simulink model "TrackingAdaptiveTaskSpace"  (R2019a)
settings: Solver=ode23  StartTime=0.0  StopTime=10  FixedStep=0.01  RelTol=1e-4
libraries: dspmtrx3 x3, dspinverses x1
(part 2 of 2)

== matlab function TrackingAdaptiveTaskSpace/MATLAB Function1 ==
  data: q1 input; aux output; q2 input; q3 input; q4 input; L1 input; L2 input; L3 input; L4 input
function aux = fcn(q1,q2,q3,q4,L1,L2,L3,L4)
%%%
aux11 = 0;
aux21 = (0.5000*(L2*L4*cos(conj(q1))*cos(conj(q1) + conj(q2) + conj(q3))*cos(q1 + q2 + q3 + q4)*conj(L1)*conj(L3)*sin(q1 + q2) - L2*L4*cos(conj(q1))*cos(conj(q1) + conj(q2) + conj(q3))*sin(q1 + q2 + q3 + q4)*cos(q1 + q2)*conj(L1)*conj(L3) + 3*L1*L4*cos(conj(q1) + conj(q2) + conj(q3) + conj(q4))*cos(conj(q1))*cos(q1 + q2 + q3 + q4)*conj(L1)*conj(L4)*sin(q1) - 3*L1*L4*cos(conj(q1) + conj(q2) + conj(q3) + conj(q4))*cos(conj(q1))*sin(q1 + q2 + q3 + q4)*conj(L1)*conj(L4)*cos(q1) + 3*L1*L4*cos(conj(q1) + conj(q2) + conj(q3) + conj(q4))*sin(conj(q1))*cos(q1 + q2 + q3 + q4)*conj(L1)*conj(L4)*cos(q1) - 3*L1*L4*sin(conj(q1) + conj(q2) + conj(q3) + conj(q4))*cos(conj(q1))*cos(q1 + q2 + q3 + q4)*conj(L1)*conj(L4)*cos(q1) + L1*L3*cos(q1 + q2 + q3)*sin(conj(q1))*sin(conj(q1) + conj(q2))*conj(L1)*conj(L2)*sin(q1) - L1*L3*sin(q1 + q2 + q3)*cos(conj(q1))*sin(conj(q1) + conj(q2))*conj(L1)*conj(L2)*sin(q1) + L1*L3*sin(q1 + q2 + q3)*sin(conj(q1))*cos(conj(q1) + conj(q2))*conj(L1)*conj(L2)*sin(q1) - L1*L3*sin(q1 + q2 + q3)*sin(conj(q1))*sin(conj(q1) + conj(q2))*conj(L1)*conj(L2)*cos(q1) + L1*L4*cos(conj(q1) + conj(q2) + conj(q3) + conj(q4))*sin(conj(q1) + conj(q2) + conj(q3))*cos(q1 + q2 + q3 + q4)*conj(L3)*conj(L4)*cos(q1) - L1*L4*sin(conj(q1) + conj(q2) + conj(q3) + conj(q4))*cos(conj(q1) + conj(q2) + conj(q3))*cos(q1 + q2 + q3 + q4)*conj(L3)*conj(L4)*cos(q1) + L1*L3*sin(q1 + q2 + q3)*cos(conj(q1) + conj(q2) + conj(q3))*sin(conj(q1) + conj(q2))*conj(L2)*conj(L3)*sin(q1) - L1*L3*sin(q1 + q2 + q3)*sin(conj(q1) + conj(q2) + conj(q3))*cos(conj(q1) + conj(q2))*conj(L2)*conj(L3)*sin(q1) + L2*L4*sin(conj(q1))*sin(conj(q1) + conj(q2) + conj(q3))*cos(q1 + q2 + q3 + q4)*conj(L1)*conj(L3)*sin(q1 + q2) - L2*L4*sin(conj(q1))*sin(conj(q1) + conj(q2) + conj(q3))*sin(q1 + q2 + q3 + q4)*cos(q1 + q2)*conj(L1)*conj(L3) + L1*L2*cos(conj(q1) + conj(q2) + conj(q3) + conj(q4))*cos(conj(q1))*cos(q1 + q2)*conj(L1)*conj(L4)*sin(q1) - L1*L2*cos(conj(q1) + conj(q2) + conj(q3) + conj(q4))*cos(conj(q1))*conj(L1)*conj(L4)*sin(q1 + q2)*cos(q1) + L1*L2*cos(conj(q1) + conj(q2) + conj(q3) + conj(q4))*sin(conj(q1))*cos(q1 + q2)*conj(L1)*conj(L4)*cos(q1) - L1*L2*sin(conj(q1) + conj(q2) + conj(q3) + conj(q4))*cos(conj(q1))*cos(q1 + q2)*conj(L1)*conj(L4)*cos(q1) + 3*L1*L4*cos(conj(q1) + conj(q2) + conj(q3) + conj(q4))*sin(conj(q1))*sin(q1 + q2 + q3 + q4)*conj(L1)*conj(L4)*sin(q1) - 3*L1*L4*sin(conj(q1) + conj(q2) + conj(q3) + conj(q4))*cos(conj(q1))*sin(q1 + q2 + q3 + q4)*conj(L1)*conj(L4)*sin(q1) + 3*L1*L4*sin(conj(q1) + conj(q2) + conj(q3) + conj(q4))*sin(conj(q1))*cos(q1 + q2 + q3 + q4)*conj(L1)*conj(L4)*sin(q1) - 3*L1*L4*sin(conj(q1) + conj(q2) + conj(q3) + conj(q4))*sin(conj(q1))*sin(q1 + q2 + q3 + q4)*conj(L1)*conj(L4)*cos(q1) + L1*L4*cos(conj(q1) + conj(q2) + conj(q3) + conj(q4))*sin(conj(q1) + conj(q2) + conj(q3))*sin(q1 + q2 + q3 + q4)*conj(L3)*conj(L4)*sin(q1) - L1*L4*sin(conj(q1) + conj(q2) + conj(q3) + conj(q4))*cos(conj(q1) + conj(q2) + conj(q3))*sin(q1 + q2 + q3 + q4)*conj(L3)*conj(L4)*sin(q1) + 2*L1*L4*cos(conj(q1))*cos(conj(q1) + conj(q2) + conj(q3))*cos(q1 + q2 + q3 + q4)*conj(L1)*conj(L3)*sin(q1) - 2*L1*L4*cos(conj(q1))*cos(conj(q1) + conj(q2) + conj(q3))*sin(q1 + q2 + q3 + q4)*conj(L1)*conj(L3)*cos(q1) - 2*L1*L4*cos(conj(q1))*sin(conj(q1) + conj(q2) + conj(q3))*cos(q1 + q2 + q3 + q4)*conj(L1)*conj(L3)*cos(q1) + 2*L1*L4*cos(conj(q1) + conj(q2) + conj(q3))*sin(conj(q1))*cos(q1 + q2 + q3 + q4)*conj(L1)*conj(L3)*cos(q1) + 2*L1*L4*cos(conj(q1) + conj(q2) + conj(q3) + conj(q4))*sin(conj(q1) + conj(q2))*cos(q1 + q2 + q3 + q4)*conj(L2)*conj(L4)*cos(q1) - 2*L1*L4*sin(conj(q1) + conj(q2) + conj(q3) + conj(q4))*cos(conj(q1) + conj(q2))*cos(q1 + q2 + q3 + q4)*conj(L2)*conj(L4)*cos(q1) + L1*L2*cos(conj(q1) + conj(q2) + conj(q3) + conj(q4))*sin(conj(q1))*conj(L1)*conj(L4)*sin(q1 + q2)*sin(q1) - L1*L2*sin(conj(q1) + conj(q2) + conj(q3) + conj(q4))*cos(conj(q1))*conj(L1)*conj(L4)*sin(q1 + q2)*sin(q1) + L1*L2*sin(conj(q1) + conj(q2) + conj(q3) + conj(q4))*sin(conj(q1))*cos(q1 + q2)*conj(L1)*conj(L4)*sin(q1) - L1*L2*sin(conj(q1) + conj(q2) + conj(q3) + conj(q4))*sin(conj(q1))*conj(L1)*conj(L4)*sin(q1 + q2)*cos(q1) - L3*L4*cos(conj(q1) + conj(q2) + conj(q3) + conj(q4))*cos(q1 + q2 + q3)*cos(conj(q1))*sin(q1 + q2 + q3 + q4)*conj(L1)*conj(L4) + L3*L4*cos(conj(q1) + conj(q2) + conj(q3) + conj(q4))*sin(q1 + q2 + q3)*cos(conj(q1))*cos(q1 + q2 + q3 + q4)*conj(L1)*conj(L4) + L1*L2*cos(conj(q1))*cos(conj(q1) + conj(q2) + conj(q3))*cos(q1 + q2)*conj(L1)*conj(L3)*sin(q1) - L1*L2*cos(conj(q1))*cos(conj(q1) + conj(q2) + conj(q3))*conj(L1)*conj(L3)*sin(q1 + q2)*cos(q1) - L1*L2*cos(conj(q1))*sin(conj(q1) + conj(q2) + conj(q3))*cos(q1 + q2)*conj(L1)*conj(L3)*cos(q1) + L1*L2*cos(conj(q1) + conj(q2) + conj(q3))*sin(conj(q1))*cos(q1 + q2)*conj(L1)*conj(L3)*cos(q1) - 2*L1*L4*cos(conj(q1))*sin(conj(q1) + conj(q2) + conj(q3))*sin(q1 + q2 + q3 + q4)*conj(L1)*conj(L3)*sin(q1) + 2*L1*L4*cos(conj(q1) + conj(q2) + conj(q3))*sin(conj(q1))*sin(q1 + q2 + q3 + q4)*conj(L1)*conj(L3)*sin(q1) + 2*L1*L4*sin(conj(q1))*sin(conj(q1) + conj(q2) + conj(q3))*cos(q1 + q2 + q3 + q4)*conj(L1)*conj(L3)*sin(q1) - 2*L1*L4*sin(conj(q1))*sin(conj(q1) + conj(q2) + conj(q3))*sin(q1 + q2 + q3 + q4)*conj(L1)*conj(L3)*cos(q1) + 2*L1*L4*cos(conj(q1) + conj(q2) + conj(q3) + conj(q4))*sin(conj(q1) + conj(q2))*sin(q1 + q2 + q3 + q4)*conj(L2)*conj(L4)*sin(q1) - 2*L1*L4*sin(conj(q1) + conj(q2) + conj(q3) + conj(q4))*cos(conj(q1) + conj(q2))*sin(q1 + q2 + q3 + q4)*conj(L2)*conj(L4)*sin(q1) + L1*L4*cos(conj(q1))*cos(conj(q1) + conj(q2))*cos(q1 + q2 + q3 + q4)*conj(L1)*conj(L2)*sin(q1) - L1*L4*cos(conj(q1))*cos(conj(q1) + conj(q2))*sin(q1 + q2 + q3 + q4)*conj(L1)*conj(L2)*cos(q1) - L1*L4*cos(conj(q1))*sin(conj(q1) + conj(q2))*cos(q1 + q2 + q3 + q4)*conj(L1)*conj(L2)*cos(q1) + L1*L4*sin(conj(q1))*cos(conj(q1) + conj(q2))*cos(q1 + q2 + q3 + q4)*conj(L1)*conj(L2)*cos(q1) + L1*L4*cos(conj(q1) + conj(q2) + conj(q3))*sin(conj(q1) + conj(q2))*cos(q1 + q2 + q3 + q4)*conj(L2)*conj(L3)*cos(q1) - L1*L4*sin(conj(q1) + conj(q2) + conj(q3))*cos(conj(q1) + conj(q2))*cos(q1 + q2 + q3 + q4)*conj(L2)*conj(L3)*cos(q1) + L2*L3*cos(conj(q1) + conj(q2) + conj(q3) + conj(q4))*cos(q1 + q2 + q3)*cos(conj(q1))*conj(L1)*conj(L4)*sin(q1 + q2) - L2*L3*cos(conj(q1) + conj(q2) + conj(q3) + conj(q4))*sin(q1 + q2 + q3)*cos(conj(q1))*cos(q1 + q2)*conj(L1)*conj(L4) - L3*L4*cos(q1 + q2 + q3)*sin(conj(q1) + conj(q2) + conj(q3) + conj(q4))*sin(conj(q1))*sin(q1 + q2 + q3 + q4)*conj(L1)*conj(L4) + L3*L4*sin(conj(q1) + conj(q2) + conj(q3) + conj(q4))*sin(q1 + q2 + q3)*sin(conj(q1))*cos(q1 + q2 + q3 + q4)*conj(L1)*conj(L4) - L1*L2*cos(conj(q1))*sin(conj(q1) + conj(q2) + conj(q3))*conj(L1)*conj(L3)*sin(q1 + q2)*sin(q1) + L1*L2*cos(conj(q1) + conj(q2) + conj(q3))*sin(conj(q1))*conj(L1)*conj(L3)*sin(q1 + q2)*sin(q1) + L1*L2*sin(conj(q1))*sin(conj(q1) + conj(q2) + conj(q3))*cos(q1 + q2)*conj(L1)*conj(L3)*sin(q1) - L1*L2*sin(conj(q1))*sin(conj(q1) + conj(q2) + conj(q3))*conj(L1)*conj(L3)*sin(q1 + q2)*cos(q1) + L1*L2*cos(conj(q1))*cos(conj(q1) + conj(q2))*cos(q1 + q2)*conj(L1)*conj(L2)*sin(q1) - L1*L2*cos(conj(q1))*cos(conj(q1) + conj(q2))*conj(L1)*conj(L2)*sin(q1 + q2)*cos(q1) - L1*L2*cos(conj(q1))*sin(conj(q1) + conj(q2))*cos(q1 + q2)*conj(L1)*conj(L2)*cos(q1) + L1*L2*sin(conj(q1))*cos(conj(q1) + conj(q2))*cos(q1 + q2)*conj(L1)*conj(L2)*cos(q1) - L1*L4*cos(conj(q1))*sin(conj(q1) + conj(q2))*sin(q1 + q2 + q3 + q4)*conj(L1)*conj(L2)*sin(q1) + L1*L4*sin(conj(q1))*cos(conj(q1) + conj(q2))*sin(q1 + q2 + q3 + q4)*conj(L1)*conj(L2)*sin(q1) + L1*L4*sin(conj(q1))*sin(conj(q1) + conj(q2))*cos(q1 + q2 + q3 + q4)*conj(L1)*conj(L2)*sin(q1) - L1*L4*sin(conj(q1))*sin(conj(q1) + conj(q2))*sin(q1 + q2 + q3 + q4)*conj(L1)*conj(L2)*cos(q1) + L1*L4*cos(conj(q1) + conj(q2) + conj(q3))*sin(conj(q1) + conj(q2))*sin(q1 + q2 + q3 + q4)*conj(L2)*conj(L3)*sin(q1) - L1*L4*sin(conj(q1) + conj(q2) + conj(q3))*cos(conj(q1) + conj(q2))*sin(q1 + q2 + q3 + q4)*conj(L2)*conj(L3)*sin(q1) + L2*L3*cos(q1 + q2 + q3)*sin(conj(q1) + conj(q2) + conj(q3) + conj(q4))*sin(conj(q1))*conj(L1)*conj(L4)*sin(q1 + q2) - L2*L3*sin(conj(q1) + conj(q2) + conj(q3) + conj(q4))*sin(q1 + q2 + q3)*sin(conj(q1))*cos(q1 + q2)*conj(L1)*conj(L4) + L2*L3*cos(q1 + q2 + q3)*cos(conj(q1))*cos(conj(q1) + conj(q2) + conj(q3))*conj(L1)*conj(L3)*sin(q1 + q2) - L2*L3*sin(q1 + q2 + q3)*cos(conj(q1))*cos(conj(q1) + conj(q2) + conj(q3))*cos(q1 + q2)*conj(L1)*conj(L3) + 2*L1*L3*cos(conj(q1) + conj(q2) + conj(q3) + conj(q4))*cos(q1 + q2 + q3)*cos(conj(q1))*conj(L1)*conj(L4)*sin(q1) + 2*L1*L3*cos(conj(q1) + conj(q2) + conj(q3) + conj(q4))*cos(q1 + q2 + q3)*sin(conj(q1))*conj(L1)*conj(L4)*cos(q1) - 2*L1*L3*cos(conj(q1) + conj(q2) + conj(q3) + conj(q4))*sin(q1 + q2 + q3)*cos(conj(q1))*conj(L1)*conj(L4)*cos(q1) - 2*L1*L3*cos(q1 + q2 + q3)*sin(conj(q1) + conj(q2) + conj(q3) + conj(q4))*cos(conj(q1))*conj(L1)*conj(L4)*cos(q1) - L1*L2*cos(conj(q1))*sin(conj(q1) + conj(q2))*conj(L1)*conj(L2)*sin(q1 + q2)*sin(q1) + L1*L2*sin(conj(q1))*cos(conj(q1) + conj(q2))*conj(L1)*conj(L2)*sin(q1 + q2)*sin(q1) + L1*L2*sin(conj(q1))*sin(conj(q1) + conj(q2))*cos(q1 + q2)*conj(L1)*conj(L2)*sin(q1) - L1*L2*sin(conj(q1))*sin(conj(q1) + conj(q2))*conj(L1)*conj(L2)*sin(q1 + q2)*cos(q1) + L2*L3*cos(q1 + q2 + q3)*sin(conj(q1))*sin(conj(q1) + conj(q2) + conj(q3))*conj(L1)*conj(L3)*sin(q1 + q2) - L2*L3*sin(q1 + q2 + q3)*sin(conj(q1))*sin(conj(q1) + conj(q2) + conj(q3))*cos(q1 + q2)*conj(L1)*conj(L3) + 2*L1*L3*cos(conj(q1) + conj(q2) + conj(q3) + conj(q4))*sin(q1 + q2 + q3)*sin(conj(q1))*conj(L1)*conj(L4)*sin(q1) + 2*L1*L3*cos(q1 + q2 + q3)*sin(conj(q1) + conj(q2) + conj(q3) + conj(q4))*sin(conj(q1))*conj(L1)*conj(L4)*sin(q1) - 2*L1*L3*sin(conj(q1) + conj(q2) + conj(q3) + conj(q4))*sin(q1 + q2 + q3)*cos(conj(q1))*conj(L1)*conj(L4)*sin(q1) - 2*L1*L3*sin(conj(q1) + conj(q2) + conj(q3) + conj(q4))*sin(q1 + q2 + q3)*sin(conj(q1))*conj(L1)*conj(L4)*cos(q1) + 2*L1*L3*cos(q1 + q2 + q3)*cos(conj(q1))*cos(conj(q1) + conj(q2) + conj(q3))*conj(L1)*conj(L3)*sin(q1) - 2*L1*L3*cos(q1 + q2 + q3)*cos(conj(q1))*sin(conj(q1) + conj(q2) + conj(q3))*conj(L1)*conj(L3)*cos(q1) + 2*L1*L3*cos(q1 + q2 + q3)*cos(conj(q1) + conj(q2) + conj(q3))*sin(conj(q1))*conj(L1)*conj(L3)*cos(q1) - 2*L1*L3*sin(q1 + q2 + q3)*cos(conj(q1))*cos(conj(q1) + conj(q2) + conj(q3))*conj(L1)*conj(L3)*cos(q1) + L1*L3*cos(conj(q1) + conj(q2) + conj(q3) + conj(q4))*cos(q1 + q2 + q3)*sin(conj(q1) + conj(q2))*conj(L2)*conj(L4)*cos(q1) - L1*L3*cos(q1 + q2 + q3)*sin(conj(q1) + conj(q2) + conj(q3) + conj(q4))*cos(conj(q1) + conj(q2))*conj(L2)*conj(L4)*cos(q1) + 2*L2*L4*cos(conj(q1) + conj(q2) + conj(q3) + conj(q4))*cos(conj(q1))*cos(q1 + q2 + q3 + q4)*conj(L1)*conj(L4)*sin(q1 + q2) - 2*L2*L4*cos(conj(q1) + conj(q2) + conj(q3) + conj(q4))*cos(conj(q1))*sin(q1 + q2 + q3 + q4)*cos(q1 + q2)*conj(L1)*conj(L4) + 2*L1*L3*cos(q1 + q2 + q3)*sin(conj(q1))*sin(conj(q1) + conj(q2) + conj(q3))*conj(L1)*conj(L3)*sin(q1) - 2*L1*L3*sin(q1 + q2 + q3)*cos(conj(q1))*sin(conj(q1) + conj(q2) + conj(q3))*conj(L1)*conj(L3)*sin(q1) + 2*L1*L3*sin(q1 + q2 + q3)*cos(conj(q1) + conj(q2) + conj(q3))*sin(conj(q1))*conj(L1)*conj(L3)*sin(q1) - 2*L1*L3*sin(q1 + q2 + q3)*sin(conj(q1))*sin(conj(q1) + conj(q2) + conj(q3))*conj(L1)*conj(L3)*cos(q1) + L1*L3*cos(conj(q1) + conj(q2) + conj(q3) + conj(q4))*sin(q1 + q2 + q3)*sin(conj(q1) + conj(q2))*conj(L2)*conj(L4)*sin(q1) - L1*L3*sin(conj(q1) + conj(q2) + conj(q3) + conj(q4))*sin(q1 + q2 + q3)*cos(conj(q1) + conj(q2))*conj(L2)*conj(L4)*sin(q1) + L1*L3*cos(q1 + q2 + q3)*cos(conj(q1))*cos(conj(q1) + conj(q2))*conj(L1)*conj(L2)*sin(q1) - L1*L3*cos(q1 + q2 + q3)*cos(conj(q1))*sin(conj(q1) + conj(q2))*conj(L1)*conj(L2)*cos(q1) + L1*L3*cos(q1 + q2 + q3)*sin(conj(q1))*cos(conj(q1) + conj(q2))*conj(L1)*conj(L2)*cos(q1) - L1*L3*sin(q1 + q2 + q3)*cos(conj(q1))*cos(conj(q1) + conj(q2))*conj(L1)*conj(L2)*cos(q1) + L1*L3*cos(q1 + q2 + q3)*cos(conj(q1) + conj(q2) + conj(q3))*sin(conj(q1) + conj(q2))*conj(L2)*conj(L3)*cos(q1) - L1*L3*cos(q1 + q2 + q3)*sin(conj(q1) + conj(q2) + conj(q3))*cos(conj(q1) + conj(q2))*conj(L2)*conj(L3)*cos(q1) + 2*L2*L4*sin(conj(q1) + conj(q2) + conj(q3) + conj(q4))*sin(conj(q1))*cos(q1 + q2 + q3 + q4)*conj(L1)*conj(L4)*sin(q1 + q2) - 2*L2*L4*sin(conj(q1) + conj(q2) + conj(q3) + conj(q4))*sin(conj(q1))*sin(q1 + q2 + q3 + q4)*cos(q1 + q2)*conj(L1)*conj(L4)))/(L1*L3*cos(q1 + q2 + q3)*sin(conj(q1))*cos(conj(q1) + conj(q2))*conj(L1)*conj(L2)*sin(q1) - L1*L3*cos(q1 + q2 + q3)*cos(conj(q1))*sin(conj(q1) + conj(q2))*conj(L1)*conj(L2)*sin(q1) + L1*L3*sin(q1 + q2 + q3)*cos(conj(q1))*sin(conj(q1) + conj(q2))*conj(L1)*conj(L2)*cos(q1) - L1*L3*sin(q1 + q2 + q3)*sin(conj(q1))*cos(conj(q1) + conj(q2))*conj(L1)*conj(L2)*cos(q1) + L1*L3*cos(q1 + q2 + q3)*cos(conj(q1) + conj(q2) + conj(q3))*sin(conj(q1) + conj(q2))*conj(L2)*conj(L3)*sin(q1) - L1*L3*cos(q1 + q2 + q3)*sin(conj(q1) + conj(q2) + conj(q3))*cos(conj(q1) + conj(q2))*conj(L2)*conj(L3)*sin(q1) - L1*L3*sin(q1 + q2 + q3)*cos(conj(q1) + conj(q2) + conj(q3))*sin(conj(q1) + conj(q2))*conj(L2)*conj(L3)*cos(q1) + L1*L3*sin(q1 + q2 + q3)*sin(conj(q1) + conj(q2) + conj(q3))*cos(conj(q1) + conj(q2))*conj(L2)*conj(L3)*cos(q1) - L2*L4*cos(conj(q1))*sin(conj(q1) + conj(q2) + conj(q3))*cos(q1 + q2 + q3 + q4)*conj(L1)*conj(L3)*sin(q1 + q2) + L2*L4*cos(conj(q1))*sin(conj(q1) + conj(q2) + conj(q3))*sin(q1 + q2 + q3 + q4)*cos(q1 + q2)*conj(L1)*conj(L3) + L2*L4*cos(conj(q1) + conj(q2) + conj(q3))*sin(conj(q1))*cos(q1 + q2 + q3 + q4)*conj(L1)*conj(L3)*sin(q1 + q2) - L2*L4*cos(conj(q1) + conj(q2) + conj(q3))*sin(conj(q1))*sin(q1 + q2 + q3 + q4)*cos(q1 + q2)*conj(L1)*conj(L3) + 3*L1*L4*cos(conj(q1) + conj(q2) + conj(q3) + conj(q4))*sin(conj(q1))*cos(q1 + q2 + q3 + q4)*conj(L1)*conj(L4)*sin(q1) - 3*L1*L4*cos(conj(q1) + conj(q2) + conj(q3) + conj(q4))*sin(conj(q1))*sin(q1 + q2 + q3 + q4)*conj(L1)*conj(L4)*cos(q1) - 3*L1*L4*sin(conj(q1) + conj(q2) + conj(q3) + conj(q4))*cos(conj(q1))*cos(q1 + q2 + q3 + q4)*conj(L1)*conj(L4)*sin(q1) + 3*L1*L4*sin(conj(q1) + conj(q2) + conj(q3) + conj(q4))*cos(conj(q1))*sin(q1 + q2 + q3 + q4)*conj(L1)*conj(L4)*cos(q1) + 4*L2*L4*cos(conj(q1) + conj(q2) + conj(q3) + conj(q4))*sin(conj(q1) + conj(q2))*cos(q1 + q2 + q3 + q4)*conj(L2)*conj(L4)*sin(q1 + q2) - 4*L2*L4*cos(conj(q1) + conj(q2) + conj(q3) + conj(q4))*sin(conj(q1) + conj(q2))*sin(q1 + q2 + q3 + q4)*cos(q1 + q2)*conj(L2)*conj(L4) - 4*L2*L4*sin(conj(q1) + conj(q2) + conj(q3) + conj(q4))*cos(conj(q1) + conj(q2))*cos(q1 + q2 + q3 + q4)*conj(L2)*conj(L4)*sin(q1 + q2) + 4*L2*L4*sin(conj(q1) + conj(q2) + conj(q3) + conj(q4))*cos(conj(q1) + conj(q2))*sin(q1 + q2 + q3 + q4)*cos(q1 + q2)*conj(L2)*conj(L4) + L1*L4*cos(conj(q1) + conj(q2) + conj(q3) + conj(q4))*sin(conj(q1) + conj(q2) + conj(q3))*cos(q1 + q2 + q3 + q4)*conj(L3)*conj(L4)*sin(q1) - L1*L4*cos(conj(q1) + conj(q2) + conj(q3) + conj(q4))*sin(conj(q1) + conj(q2) + conj(q3))*sin(q1 + q2 + q3 + q4)*conj(L3)*conj(L4)*cos(q1) - L1*L4*sin(conj(q1) + conj(q2) + conj(q3) + conj(q4))*cos(conj(q1) + conj(q2) + conj(q3))*cos(q1 + q2 + q3 + q4)*conj(L3)*conj(L4)*sin(q1) + L1*L4*sin(conj(q1) + conj(q2) + conj(q3) + conj(q4))*cos(conj(q1) + conj(q2) + conj(q3))*sin(q1 + q2 + q3 + q4)*conj(L3)*conj(L4)*cos(q1) + L1*L2*cos(conj(q1) + conj(q2) + conj(q3) + conj(q4))*sin(conj(q1))*cos(q1 + q2)*conj(L1)*conj(L4)*sin(q1) - L1*L2*cos(conj(q1) + conj(q2) + conj(q3) + conj(q4))*sin(conj(q1))*conj(L1)*conj(L4)*sin(q1 + q2)*cos(q1) - L1*L2*sin(conj(q1) + conj(q2) + conj(q3) + conj(q4))*cos(conj(q1))*cos(q1 + q2)*conj(L1)*conj(L4)*sin(q1) + L1*L2*sin(conj(q1) + conj(q2) + conj(q3) + conj(q4))*cos(conj(q1))*conj(L1)*conj(L4)*sin(q1 + q2)*cos(q1) - 2*L1*L4*cos(conj(q1))*sin(conj(q1) + conj(q2) + conj(q3))*cos(q1 + q2 + q3 + q4)*conj(L1)*conj(L3)*sin(q1) + 2*L1*L4*cos(conj(q1))*sin(conj(q1) + conj(q2) + conj(q3))*sin(q1 + q2 + q3 + q4)*conj(L1)*conj(L3)*cos(q1) + 2*L1*L4*cos(conj(q1) + conj(q2) + conj(q3))*sin(conj(q1))*cos(q1 + q2 + q3 + q4)*conj(L1)*conj(L3)*sin(q1) - 2*L1*L4*cos(conj(q1) + conj(q2) + conj(q3))*sin(conj(q1))*sin(q1 + q2 + q3 + q4)*conj(L1)*conj(L3)*cos(q1) + 2*L2*L4*cos(conj(q1) + conj(q2) + conj(q3))*sin(conj(q1) + conj(q2))*cos(q1 + q2 + q3 + q4)*conj(L2)*conj(L3)*sin(q1 + q2) - 2*L2*L4*cos(conj(q1) + conj(q2) + conj(q3))*sin(conj(q1) + conj(q2))*sin(q1 + q2 + q3 + q4)*cos(q1 + q2)*conj(L2)*conj(L3) - 2*L2*L4*sin(conj(q1) + conj(q2) + conj(q3))*cos(conj(q1) + conj(q2))*cos(q1 + q2 + q3 + q4)*conj(L2)*conj(L3)*sin(q1 + q2) + 2*L2*L4*sin(conj(q1) + conj(q2) + conj(q3))*cos(conj(q1) + conj(q2))*sin(q1 + q2 + q3 + q4)*cos(q1 + q2)*conj(L2)*conj(L3) + 2*L1*L4*cos(conj(q1) + conj(q2) + conj(q3) + conj(q4))*sin(conj(q1) + conj(q2))*cos(q1 + q2 + q3 + q4)*conj(L2)*conj(L4)*sin(q1) - 2*L1*L4*cos(conj(q1) + conj(q2) + conj(q3) + conj(q4))*sin(conj(q1) + conj(q2))*sin(q1 + q2 + q3 + q4)*conj(L2)*conj(L4)*cos(q1) - 2*L1*L4*sin(conj(q1) + conj(q2) + conj(q3) + conj(q4))*cos(conj(q1) + conj(q2))*cos(q1 + q2 + q3 + q4)*conj(L2)*conj(L4)*sin(q1) + 2*L1*L4*sin(conj(q1) + conj(q2) + conj(q3) + conj(q4))*cos(conj(q1) + conj(q2))*sin(q1 + q2 + q3 + q4)*conj(L2)*conj(L4)*cos(q1) - L3*L4*cos(conj(q1) + conj(q2) + conj(q3) + conj(q4))*cos(q1 + q2 + q3)*sin(conj(q1))*sin(q1 + q2 + q3 + q4)*conj(L1)*conj(L4) + L3*L4*cos(conj(q1) + conj(q2) + conj(q3) + conj(q4))*sin(q1 + q2 + q3)*sin(conj(q1))*cos(q1 + q2 + q3 + q4)*conj(L1)*conj(L4) + L3*L4*cos(q1 + q2 + q3)*sin(conj(q1) + conj(q2) + conj(q3) + conj(q4))*cos(conj(q1))*sin(q1 + q2 + q3 + q4)*conj(L1)*conj(L4) - L3*L4*sin(conj(q1) + conj(q2) + conj(q3) + conj(q4))*sin(q1 + q2 + q3)*cos(conj(q1))*cos(q1 + q2 + q3 + q4)*conj(L1)*conj(L4) - L1*L2*cos(conj(q1))*sin(conj(q1) + conj(q2) + conj(q3))*cos(q1 + q2)*conj(L1)*conj(L3)*sin(q1) + L1*L2*cos(conj(q1))*sin(conj(q1) + conj(q2) + conj(q3))*conj(L1)*conj(L3)*sin(q1 + q2)*cos(q1) + L1*L2*cos(conj(q1) + conj(q2) + conj(q3))*sin(conj(q1))*cos(q1 + q2)*conj(L1)*conj(L3)*sin(q1) - L1*L2*cos(conj(q1) + conj(q2) + conj(q3))*sin(conj(q1))*conj(L1)*conj(L3)*sin(q1 + q2)*cos(q1) - 3*L3*L4*cos(conj(q1) + conj(q2) + conj(q3) + conj(q4))*cos(q1 + q2 + q3)*sin(conj(q1) + conj(q2) + conj(q3))*sin(q1 + q2 + q3 + q4)*conj(L3)*conj(L4) + 3*L3*L4*cos(conj(q1) + conj(q2) + conj(q3) + conj(q4))*sin(q1 + q2 + q3)*sin(conj(q1) + conj(q2) + conj(q3))*cos(q1 + q2 + q3 + q4)*conj(L3)*conj(L4) + 3*L3*L4*cos(q1 + q2 + q3)*sin(conj(q1) + conj(q2) + conj(q3) + conj(q4))*cos(conj(q1) + conj(q2) + conj(q3))*sin(q1 + q2 + q3 + q4)*conj(L3)*conj(L4) - 3*L3*L4*sin(conj(q1) + conj(q2) + conj(q3) + conj(q4))*sin(q1 + q2 + q3)*cos(conj(q1) + conj(q2) + conj(q3))*cos(q1 + q2 + q3 + q4)*conj(L3)*conj(L4) - L1*L4*cos(conj(q1))*sin(conj(q1) + conj(q2))*cos(q1 + q2 + q3 + q4)*conj(L1)*conj(L2)*sin(q1) + L1*L4*cos(conj(q1))*sin(conj(q1) + conj(q2))*sin(q1 + q2 + q3 + q4)*conj(L1)*conj(L2)*cos(q1) + L1*L4*sin(conj(q1))*cos(conj(q1) + conj(q2))*cos(q1 + q2 + q3 + q4)*conj(L1)*conj(L2)*sin(q1) - L1*L4*sin(conj(q1))*cos(conj(q1) + conj(q2))*sin(q1 + q2 + q3 + q4)*conj(L1)*conj(L2)*cos(q1) + L1*L4*cos(conj(q1) + conj(q2) + conj(q3))*sin(conj(q1) + conj(q2))*cos(q1 + q2 + q3 + q4)*conj(L2)*conj(L3)*sin(q1) - L1*L4*cos(conj(q1) + conj(q2) + conj(q3))*sin(conj(q1) + conj(q2))*sin(q1 + q2 + q3 + q4)*conj(L2)*conj(L3)*cos(q1) - L1*L4*sin(conj(q1) + conj(q2) + conj(q3))*cos(conj(q1) + conj(q2))*cos(q1 + q2 + q3 + q4)*conj(L2)*conj(L3)*sin(q1) + L1*L4*sin(conj(q1) + conj(q2) + conj(q3))*cos(conj(q1) + conj(q2))*sin(q1 + q2 + q3 + q4)*conj(L2)*conj(L3)*cos(q1) + L2*L3*cos(conj(q1) + conj(q2) + conj(q3) + conj(q4))*cos(q1 + q2 + q3)*sin(conj(q1))*conj(L1)*conj(L4)*sin(q1 + q2) - L2*L3*cos(conj(q1) + conj(q2) + conj(q3) + conj(q4))*sin(q1 + q2 + q3)*sin(conj(q1))*cos(q1 + q2)*conj(L1)*conj(L4) - L2*L3*cos(q1 + q2 + q3)*sin(conj(q1) + conj(q2) + conj(q3) + conj(q4))*cos(conj(q1))*conj(L1)*conj(L4)*sin(q1 + q2) + L2*L3*sin(conj(q1) + conj(q2) + conj(q3) + conj(q4))*sin(q1 + q2 + q3)*cos(conj(q1))*cos(q1 + q2)*conj(L1)*conj(L4) - L1*L2*cos(conj(q1))*sin(conj(q1) + conj(q2))*cos(q1 + q2)*conj(L1)*conj(L2)*sin(q1) + L1*L2*cos(conj(q1))*sin(conj(q1) + conj(q2))*conj(L1)*conj(L2)*sin(q1 + q2)*cos(q1) + L1*L2*sin(conj(q1))*cos(conj(q1) + conj(q2))*cos(q1 + q2)*conj(L1)*conj(L2)*sin(q1) - L1*L2*sin(conj(q1))*cos(conj(q1) + conj(q2))*conj(L1)*conj(L2)*sin(q1 + q2)*cos(q1) - 2*L3*L4*cos(conj(q1) + conj(q2) + conj(q3) + conj(q4))*cos(q1 + q2 + q3)*sin(conj(q1) + conj(q2))*sin(q1 + q2 + q3 + q4)*conj(L2)*conj(L4) + 2*L3*L4*cos(conj(q1) + conj(q2) + conj(q3) + conj(q4))*sin(q1 + q2 + q3)*sin(conj(q1) + conj(q2))*cos(q1 + q2 + q3 + q4)*conj(L2)*conj(L4) + 2*L3*L4*cos(q1 + q2 + q3)*sin(conj(q1) + conj(q2) + conj(q3) + conj(q4))*cos(conj(q1) + conj(q2))*sin(q1 + q2 + q3 + q4)*conj(L2)*conj(L4) - 2*L3*L4*sin(conj(q1) + conj(q2) + conj(q3) + conj(q4))*sin(q1 + q2 + q3)*cos(conj(q1) + conj(q2))*cos(q1 + q2 + q3 + q4)*conj(L2)*conj(L4) - L2*L3*cos(q1 + q2 + q3)*cos(conj(q1))*sin(conj(q1) + conj(q2) + conj(q3))*conj(L1)*conj(L3)*sin(q1 + q2) + L2*L3*cos(q1 + q2 + q3)*cos(conj(q1) + conj(q2) + conj(q3))*sin(conj(q1))*conj(L1)*conj(L3)*sin(q1 + q2) + L2*L3*sin(q1 + q2 + q3)*cos(conj(q1))*sin(conj(q1) + conj(q2) + conj(q3))*cos(q1 + q2)*conj(L1)*conj(L3) - L2*L3*sin(q1 + q2 + q3)*cos(conj(q1) + conj(q2) + conj(q3))*sin(conj(q1))*cos(q1 + q2)*conj(L1)*conj(L3) + 2*L1*L3*cos(conj(q1) + conj(q2) + conj(q3) + conj(q4))*cos(q1 + q2 + q3)*sin(conj(q1))*conj(L1)*conj(L4)*sin(q1) - 2*L1*L3*cos(conj(q1) + conj(q2) + conj(q3) + conj(q4))*sin(q1 + q2 + q3)*sin(conj(q1))*conj(L1)*conj(L4)*cos(q1) - 2*L1*L3*cos(q1 + q2 + q3)*sin(conj(q1) + conj(q2) + conj(q3) + conj(q4))*cos(conj(q1))*conj(L1)*conj(L4)*sin(q1) + 2*L1*L3*sin(conj(q1) + conj(q2) + conj(q3) + conj(q4))*sin(q1 + q2 + q3)*cos(conj(q1))*conj(L1)*conj(L4)*cos(q1) + 2*L2*L3*cos(conj(q1) + conj(q2) + conj(q3) + conj(q4))*cos(q1 + q2 + q3)*sin(conj(q1) + conj(q2))*conj(L2)*conj(L4)*sin(q1 + q2) - 2*L2*L3*cos(conj(q1) + conj(q2) + conj(q3) + conj(q4))*sin(q1 + q2 + q3)*sin(conj(q1) + conj(q2))*cos(q1 + q2)*conj(L2)*conj(L4) - 2*L2*L3*cos(q1 + q2 + q3)*sin(conj(q1) + conj(q2) + conj(q3) + conj(q4))*cos(conj(q1) + conj(q2))*conj(L2)*conj(L4)*sin(q1 + q2) + 2*L2*L3*sin(conj(q1) + conj(q2) + conj(q3) + conj(q4))*sin(q1 + q2 + q3)*cos(conj(q1) + conj(q2))*cos(q1 + q2)*conj(L2)*conj(L4) - 2*L1*L3*cos(q1 + q2 + q3)*cos(conj(q1))*sin(conj(q1) + conj(q2) + conj(q3))*conj(L1)*conj(L3)*sin(q1) + 2*L1*L3*cos(q1 + q2 + q3)*cos(conj(q1) + conj(q2) + conj(q3))*sin(conj(q1))*conj(L1)*conj(L3)*sin(q1) + 2*L1*L3*sin(q1 + q2 + q3)*cos(conj(q1))*sin(conj(q1) + conj(q2) + conj(q3))*conj(L1)*conj(L3)*cos(q1) - 2*L1*L3*sin(q1 + q2 + q3)*cos(conj(q1) + conj(q2) + conj(q3))*sin(conj(q1))*conj(L1)*conj(L3)*cos(q1) + 2*L2*L3*cos(q1 + q2 + q3)*cos(conj(q1) + conj(q2) + conj(q3))*sin(conj(q1) + conj(q2))*conj(L2)*conj(L3)*sin(q1 + q2) - 2*L2*L3*cos(q1 + q2 + q3)*sin(conj(q1) + conj(q2) + conj(q3))*cos(conj(q1) + conj(q2))*conj(L2)*conj(L3)*sin(q1 + q2) - 2*L2*L3*sin(q1 + q2 + q3)*cos(conj(q1) + conj(q2) + conj(q3))*sin(conj(q1) + conj(q2))*cos(q1 + q2)*conj(L2)*conj(L3) + 2*L2*L3*sin(q1 + q2 + q3)*sin(conj(q1) + conj(q2) + conj(q3))*cos(conj(q1) + conj(q2))*cos(q1 + q2)*conj(L2)*conj(L3) + L1*L3*cos(conj(q1) + conj(q2) + conj(q3) + conj(q4))*cos(q1 + q2 + q3)*sin(conj(q1) + conj(q2))*conj(L2)*conj(L4)*sin(q1) - L1*L3*cos(conj(q1) + conj(q2) + conj(q3) + conj(q4))*sin(q1 + q2 + q3)*sin(conj(q1) + conj(q2))*conj(L2)*conj(L4)*cos(q1) - L1*L3*cos(q1 + q2 + q3)*sin(conj(q1) + conj(q2) + conj(q3) + conj(q4))*cos(conj(q1) + conj(q2))*conj(L2)*conj(L4)*sin(q1) + L1*L3*sin(conj(q1) + conj(q2) + conj(q3) + conj(q4))*sin(q1 + q2 + q3)*cos(conj(q1) + conj(q2))*conj(L2)*conj(L4)*cos(q1) + 2*L2*L4*cos(conj(q1) + conj(q2) + conj(q3) + conj(q4))*sin(conj(q1))*cos(q1 + q2 + q3 + q4)*conj(L1)*conj(L4)*sin(q1 + q2) - 2*L2*L4*cos(conj(q1) + conj(q2) + conj(q3) + conj(q4))*sin(conj(q1))*sin(q1 + q2 + q3 + q4)*cos(q1 + q2)*conj(L1)*conj(L4) - 2*L2*L4*sin(conj(q1) + conj(q2) + conj(q3) + conj(q4))*cos(conj(q1))*cos(q1 + q2 + q3 + q4)*conj(L1)*conj(L4)*sin(q1 + q2) + 2*L2*L4*sin(conj(q1) + conj(q2) + conj(q3) + conj(q4))*cos(conj(q1))*sin(q1 + q2 + q3 + q4)*cos(q1 + q2)*conj(L1)*conj(L4) + 2*L2*L4*cos(conj(q1) + conj(q2) + conj(q3) + conj(q4))*sin(conj(q1) + conj(q2) + conj(q3))*cos(q1 + q2 + q3 + q4)*conj(L3)*conj(L4)*sin(q1 + q2) - 2*L2*L4*cos(conj(q1) + conj(q2) + conj(q3) + conj(q4))*sin(conj(q1) + conj(q2) + conj(q3))*sin(q1 + q2 + q3 + q4)*cos(q1 + q2)*conj(L3)*conj(L4) - 2*L2*L4*sin(conj(q1) + conj(q2) + conj(q3) + conj(q4))*cos(conj(q1) + conj(q2) + conj(q3))*cos(q1 + q2 + q3 + q4)*conj(L3)*conj(L4)*sin(q1 + q2) + 2*L2*L4*sin(conj(q1) + conj(q2) + conj(q3) + conj(q4))*cos(conj(q1) + conj(q2) + conj(q3))*sin(q1 + q2 + q3 + q4)*cos(q1 + q2)*conj(L3)*conj(L4))^0.5000;
aux31 = (0.5000*(2*L2*L4*cos(conj(q1) + conj(q2) + conj(q3) + conj(q4))*sin(conj(q1) + conj(q2) + conj(q3))*sin(q1 + q2 + q3 + q4)*conj(L3)*conj(L4)*sin(q1 + q2) - 2*L2*L4*sin(conj(q1) + conj(q2) + conj(q3) + conj(q4))*cos(conj(q1) + conj(q2) + conj(q3))*sin(q1 + q2 + q3 + q4)*conj(L3)*conj(L4)*sin(q1 + q2) + L2*L4*cos(conj(q1))*cos(conj(q1) + conj(q2) + conj(q3))*cos(q1 + q2 + q3 + q4)*conj(L1)*conj(L3)*sin(q1 + q2) - L2*L4*cos(conj(q1))*cos(conj(q1) + conj(q2) + conj(q3))*sin(q1 + q2 + q3 + q4)*cos(q1 + q2)*conj(L1)*conj(L3) - L2*L4*cos(conj(q1))*sin(conj(q1) + conj(q2) + conj(q3))*cos(q1 + q2 + q3 + q4)*cos(q1 + q2)*conj(L1)*conj(L3) + L2*L4*cos(conj(q1) + conj(q2) + conj(q3))*sin(conj(q1))*cos(q1 + q2 + q3 + q4)*cos(q1 + q2)*conj(L1)*conj(L3) + 3*L1*L4*cos(conj(q1) + conj(q2) + conj(q3) + conj(q4))*cos(conj(q1))*cos(q1 + q2 + q3 + q4)*conj(L1)*conj(L4)*sin(q1) - 3*L1*L4*cos(conj(q1) + conj(q2) + conj(q3) + conj(q4))*cos(conj(q1))*sin(q1 + q2 + q3 + q4)*conj(L1)*conj(L4)*cos(q1) + 3*L1*L4*cos(conj(q1) + conj(q2) + conj(q3) + conj(q4))*sin(conj(q1))*cos(q1 + q2 + q3 + q4)*conj(L1)*conj(L4)*cos(q1) - 3*L1*L4*sin(conj(q1) + conj(q2) + conj(q3) + conj(q4))*cos(conj(q1))*cos(q1 + q2 + q3 + q4)*conj(L1)*conj(L4)*cos(q1) + 4*L2*L4*cos(conj(q1) + conj(q2) + conj(q3) + conj(q4))*cos(conj(q1) + conj(q2))*cos(q1 + q2 + q3 + q4)*conj(L2)*conj(L4)*sin(q1 + q2) - 4*L2*L4*cos(conj(q1) + conj(q2) + conj(q3) + conj(q4))*cos(conj(q1) + conj(q2))*sin(q1 + q2 + q3 + q4)*cos(q1 + q2)*conj(L2)*conj(L4) + 4*L2*L4*cos(conj(q1) + conj(q2) + conj(q3) + conj(q4))*sin(conj(q1) + conj(q2))*cos(q1 + q2 + q3 + q4)*cos(q1 + q2)*conj(L2)*conj(L4) - 4*L2*L4*sin(conj(q1) + conj(q2) + conj(q3) + conj(q4))*cos(conj(q1) + conj(q2))*cos(q1 + q2 + q3 + q4)*cos(q1 + q2)*conj(L2)*conj(L4) - L1*L3*sin(q1 + q2 + q3)*cos(conj(q1))*sin(conj(q1) + conj(q2))*conj(L1)*conj(L2)*sin(q1) + L1*L3*sin(q1 + q2 + q3)*sin(conj(q1))*cos(conj(q1) + conj(q2))*conj(L1)*conj(L2)*sin(q1) + L1*L4*cos(conj(q1) + conj(q2) + conj(q3) + conj(q4))*sin(conj(q1) + conj(q2) + conj(q3))*cos(q1 + q2 + q3 + q4)*conj(L3)*conj(L4)*cos(q1) - L1*L4*sin(conj(q1) + conj(q2) + conj(q3) + conj(q4))*cos(conj(q1) + conj(q2) + conj(q3))*cos(q1 + q2 + q3 + q4)*conj(L3)*conj(L4)*cos(q1) + L1*L3*cos(q1 + q2 + q3)*sin(conj(q1) + conj(q2) + conj(q3))*sin(conj(q1) + conj(q2))*conj(L2)*conj(L3)*sin(q1) + L1*L3*sin(q1 + q2 + q3)*cos(conj(q1) + conj(q2) + conj(q3))*sin(conj(q1) + conj(q2))*conj(L2)*conj(L3)*sin(q1) - L1*L3*sin(q1 + q2 + q3)*sin(conj(q1) + conj(q2) + conj(q3))*cos(conj(q1) + conj(q2))*conj(L2)*conj(L3)*sin(q1) - L1*L3*sin(q1 + q2 + q3)*sin(conj(q1) + conj(q2) + conj(q3))*sin(conj(q1) + conj(q2))*conj(L2)*conj(L3)*cos(q1) - L2*L4*cos(conj(q1))*sin(conj(q1) + conj(q2) + conj(q3))*sin(q1 + q2 + q3 + q4)*conj(L1)*conj(L3)*sin(q1 + q2) + L2*L4*cos(conj(q1) + conj(q2) + conj(q3))*sin(conj(q1))*sin(q1 + q2 + q3 + q4)*conj(L1)*conj(L3)*sin(q1 + q2) + L2*L4*sin(conj(q1))*sin(conj(q1) + conj(q2) + conj(q3))*cos(q1 + q2 + q3 + q4)*conj(L1)*conj(L3)*sin(q1 + q2) - L2*L4*sin(conj(q1))*sin(conj(q1) + conj(q2) + conj(q3))*sin(q1 + q2 + q3 + q4)*cos(q1 + q2)*conj(L1)*conj(L3) + L1*L2*cos(conj(q1) + conj(q2) + conj(q3) + conj(q4))*cos(conj(q1))*cos(q1 + q2)*conj(L1)*conj(L4)*sin(q1) - L1*L2*cos(conj(q1) + conj(q2) + conj(q3) + conj(q4))*cos(conj(q1))*conj(L1)*conj(L4)*sin(q1 + q2)*cos(q1) + 3*L1*L4*cos(conj(q1) + conj(q2) + conj(q3) + conj(q4))*sin(conj(q1))*sin(q1 + q2 + q3 + q4)*conj(L1)*conj(L4)*sin(q1) - 3*L1*L4*sin(conj(q1) + conj(q2) + conj(q3) + conj(q4))*cos(conj(q1))*sin(q1 + q2 + q3 + q4)*conj(L1)*conj(L4)*sin(q1) + 3*L1*L4*sin(conj(q1) + conj(q2) + conj(q3) + conj(q4))*sin(conj(q1))*cos(q1 + q2 + q3 + q4)*conj(L1)*conj(L4)*sin(q1) - 3*L1*L4*sin(conj(q1) + conj(q2) + conj(q3) + conj(q4))*sin(conj(q1))*sin(q1 + q2 + q3 + q4)*conj(L1)*conj(L4)*cos(q1) + 4*L2*L4*cos(conj(q1) + conj(q2) + conj(q3) + conj(q4))*sin(conj(q1) + conj(q2))*sin(q1 + q2 + q3 + q4)*conj(L2)*conj(L4)*sin(q1 + q2) - 4*L2*L4*sin(conj(q1) + conj(q2) + conj(q3) + conj(q4))*cos(conj(q1) + conj(q2))*sin(q1 + q2 + q3 + q4)*conj(L2)*conj(L4)*sin(q1 + q2) + 4*L2*L4*sin(conj(q1) + conj(q2) + conj(q3) + conj(q4))*sin(conj(q1) + conj(q2))*cos(q1 + q2 + q3 + q4)*conj(L2)*conj(L4)*sin(q1 + q2) - 4*L2*L4*sin(conj(q1) + conj(q2) + conj(q3) + conj(q4))*sin(conj(q1) + conj(q2))*sin(q1 + q2 + q3 + q4)*cos(q1 + q2)*conj(L2)*conj(L4) + L1*L4*cos(conj(q1) + conj(q2) + conj(q3) + conj(q4))*sin(conj(q1) + conj(q2) + conj(q3))*sin(q1 + q2 + q3 + q4)*conj(L3)*conj(L4)*sin(q1) - L1*L4*sin(conj(q1) + conj(q2) + conj(q3) + conj(q4))*cos(conj(q1) + conj(q2) + conj(q3))*sin(q1 + q2 + q3 + q4)*conj(L3)*conj(L4)*sin(q1) + 2*L1*L4*cos(conj(q1))*cos(conj(q1) + conj(q2) + conj(q3))*cos(q1 + q2 + q3 + q4)*conj(L1)*conj(L3)*sin(q1) - 2*L1*L4*cos(conj(q1))*cos(conj(q1) + conj(q2) + conj(q3))*sin(q1 + q2 + q3 + q4)*conj(L1)*conj(L3)*cos(q1) - 2*L1*L4*cos(conj(q1))*sin(conj(q1) + conj(q2) + conj(q3))*cos(q1 + q2 + q3 + q4)*conj(L1)*conj(L3)*cos(q1) + 2*L1*L4*cos(conj(q1) + conj(q2) + conj(q3))*sin(conj(q1))*cos(q1 + q2 + q3 + q4)*conj(L1)*conj(L3)*cos(q1) + 2*L2*L4*cos(conj(q1) + conj(q2) + conj(q3))*cos(conj(q1) + conj(q2))*cos(q1 + q2 + q3 + q4)*conj(L2)*conj(L3)*sin(q1 + q2) - 2*L2*L4*cos(conj(q1) + conj(q2) + conj(q3))*cos(conj(q1) + conj(q2))*sin(q1 + q2 + q3 + q4)*cos(q1 + q2)*conj(L2)*conj(L3) + 2*L2*L4*cos(conj(q1) + conj(q2) + conj(q3))*sin(conj(q1) + conj(q2))*cos(q1 + q2 + q3 + q4)*cos(q1 + q2)*conj(L2)*conj(L3) - 2*L2*L4*sin(conj(q1) + conj(q2) + conj(q3))*cos(conj(q1) + conj(q2))*cos(q1 + q2 + q3 + q4)*cos(q1 + q2)*conj(L2)*conj(L3) + 2*L1*L4*cos(conj(q1) + conj(q2) + conj(q3) + conj(q4))*cos(conj(q1) + conj(q2))*cos(q1 + q2 + q3 + q4)*conj(L2)*conj(L4)*sin(q1) - 2*L1*L4*cos(conj(q1) + conj(q2) + conj(q3) + conj(q4))*cos(conj(q1) + conj(q2))*sin(q1 + q2 + q3 + q4)*conj(L2)*conj(L4)*cos(q1) + 2*L1*L4*cos(conj(q1) + conj(q2) + conj(q3) + conj(q4))*sin(conj(q1) + conj(q2))*cos(q1 + q2 + q3 + q4)*conj(L2)*conj(L4)*cos(q1) - 2*L1*L4*sin(conj(q1) + conj(q2) + conj(q3) + conj(q4))*cos(conj(q1) + conj(q2))*cos(q1 + q2 + q3 + q4)*conj(L2)*conj(L4)*cos(q1) + L1*L2*sin(conj(q1) + conj(q2) + conj(q3) + conj(q4))*sin(conj(q1))*cos(q1 + q2)*conj(L1)*conj(L4)*sin(q1) - L1*L2*sin(conj(q1) + conj(q2) + conj(q3) + conj(q4))*sin(conj(q1))*conj(L1)*conj(L4)*sin(q1 + q2)*cos(q1) - L3*L4*cos(conj(q1) + conj(q2) + conj(q3) + conj(q4))*cos(q1 + q2 + q3)*cos(conj(q1))*sin(q1 + q2 + q3 + q4)*conj(L1)*conj(L4) + L3*L4*cos(conj(q1) + conj(q2) + conj(q3) + conj(q4))*sin(q1 + q2 + q3)*cos(conj(q1))*cos(q1 + q2 + q3 + q4)*conj(L1)*conj(L4) + L1*L2*cos(conj(q1))*cos(conj(q1) + conj(q2) + conj(q3))*cos(q1 + q2)*conj(L1)*conj(L3)*sin(q1) - L1*L2*cos(conj(q1))*cos(conj(q1) + conj(q2) + conj(q3))*conj(L1)*conj(L3)*sin(q1 + q2)*cos(q1) - 2*L1*L4*cos(conj(q1))*sin(conj(q1) + conj(q2) + conj(q3))*sin(q1 + q2 + q3 + q4)*conj(L1)*conj(L3)*sin(q1) + 2*L1*L4*cos(conj(q1) + conj(q2) + conj(q3))*sin(conj(q1))*sin(q1 + q2 + q3 + q4)*conj(L1)*conj(L3)*sin(q1) + 2*L1*L4*sin(conj(q1))*sin(conj(q1) + conj(q2) + conj(q3))*cos(q1 + q2 + q3 + q4)*conj(L1)*conj(L3)*sin(q1) - 2*L1*L4*sin(conj(q1))*sin(conj(q1) + conj(q2) + conj(q3))*sin(q1 + q2 + q3 + q4)*conj(L1)*conj(L3)*cos(q1) + 2*L2*L4*cos(conj(q1) + conj(q2) + conj(q3))*sin(conj(q1) + conj(q2))*sin(q1 + q2 + q3 + q4)*conj(L2)*conj(L3)*sin(q1 + q2) - 2*L2*L4*sin(conj(q1) + conj(q2) + conj(q3))*cos(conj(q1) + conj(q2))*sin(q1 + q2 + q3 + q4)*conj(L2)*conj(L3)*sin(q1 + q2) + 2*L2*L4*sin(conj(q1) + conj(q2) + conj(q3))*sin(conj(q1) + conj(q2))*cos(q1 + q2 + q3 + q4)*conj(L2)*conj(L3)*sin(q1 + q2) - 2*L2*L4*sin(conj(q1) + conj(q2) + conj(q3))*sin(conj(q1) + conj(q2))*sin(q1 + q2 + q3 + q4)*cos(q1 + q2)*conj(L2)*conj(L3) + 2*L1*L4*cos(conj(q1) + conj(q2) + conj(q3) + conj(q4))*sin(conj(q1) + conj(q2))*sin(q1 + q2 + q3 + q4)*conj(L2)*conj(L4)*sin(q1) - 2*L1*L4*sin(conj(q1) + conj(q2) + conj(q3) + conj(q4))*cos(conj(q1) + conj(q2))*sin(q1 + q2 + q3 + q4)*conj(L2)*conj(L4)*sin(q1) + 2*L1*L4*sin(conj(q1) + conj(q2) + conj(q3) + conj(q4))*sin(conj(q1) + conj(q2))*cos(q1 + q2 + q3 + q4)*conj(L2)*conj(L4)*sin(q1) - 2*L1*L4*sin(conj(q1) + conj(q2) + conj(q3) + conj(q4))*sin(conj(q1) + conj(q2))*sin(q1 + q2 + q3 + q4)*conj(L2)*conj(L4)*cos(q1) - L1*L4*cos(conj(q1))*sin(conj(q1) + conj(q2))*cos(q1 + q2 + q3 + q4)*conj(L1)*conj(L2)*cos(q1) + L1*L4*sin(conj(q1))*cos(conj(q1) + conj(q2))*cos(q1 + q2 + q3 + q4)*conj(L1)*conj(L2)*cos(q1) + L1*L4*cos(conj(q1) + conj(q2) + conj(q3))*cos(conj(q1) + conj(q2))*cos(q1 + q2 + q3 + q4)*conj(L2)*conj(L3)*sin(q1) - L1*L4*cos(conj(q1) + conj(q2) + conj(q3))*cos(conj(q1) + conj(q2))*sin(q1 + q2 + q3 + q4)*conj(L2)*conj(L3)*cos(q1) + L1*L4*cos(conj(q1) + conj(q2) + conj(q3))*sin(conj(q1) + conj(q2))*cos(q1 + q2 + q3 + q4)*conj(L2)*conj(L3)*cos(q1) - L1*L4*sin(conj(q1) + conj(q2) + conj(q3))*cos(conj(q1) + conj(q2))*cos(q1 + q2 + q3 + q4)*conj(L2)*conj(L3)*cos(q1) + L2*L3*cos(conj(q1) + conj(q2) + conj(q3) + conj(q4))*cos(q1 + q2 + q3)*cos(conj(q1))*conj(L1)*conj(L4)*sin(q1 + q2) + L2*L3*cos(conj(q1) + conj(q2) + conj(q3) + conj(q4))*cos(q1 + q2 + q3)*sin(conj(q1))*cos(q1 + q2)*conj(L1)*conj(L4) - L2*L3*cos(conj(q1) + conj(q2) + conj(q3) + conj(q4))*sin(q1 + q2 + q3)*cos(conj(q1))*cos(q1 + q2)*conj(L1)*conj(L4) - L2*L3*cos(q1 + q2 + q3)*sin(conj(q1) + conj(q2) + conj(q3) + conj(q4))*cos(conj(q1))*cos(q1 + q2)*conj(L1)*conj(L4) - L3*L4*cos(q1 + q2 + q3)*sin(conj(q1) + conj(q2) + conj(q3) + conj(q4))*sin(conj(q1))*sin(q1 + q2 + q3 + q4)*conj(L1)*conj(L4) + L3*L4*sin(conj(q1) + conj(q2) + conj(q3) + conj(q4))*sin(q1 + q2 + q3)*sin(conj(q1))*cos(q1 + q2 + q3 + q4)*conj(L1)*conj(L4) + L1*L2*sin(conj(q1))*sin(conj(q1) + conj(q2) + conj(q3))*cos(q1 + q2)*conj(L1)*conj(L3)*sin(q1) - L1*L2*sin(conj(q1))*sin(conj(q1) + conj(q2) + conj(q3))*conj(L1)*conj(L3)*sin(q1 + q2)*cos(q1) - 2*L3*L4*cos(conj(q1) + conj(q2) + conj(q3) + conj(q4))*cos(q1 + q2 + q3)*cos(conj(q1) + conj(q2))*sin(q1 + q2 + q3 + q4)*conj(L2)*conj(L4) + 2*L3*L4*cos(conj(q1) + conj(q2) + conj(q3) + conj(q4))*sin(q1 + q2 + q3)*cos(conj(q1) + conj(q2))*cos(q1 + q2 + q3 + q4)*conj(L2)*conj(L4) - L1*L4*cos(conj(q1))*sin(conj(q1) + conj(q2))*sin(q1 + q2 + q3 + q4)*conj(L1)*conj(L2)*sin(q1) + L1*L4*sin(conj(q1))*cos(conj(q1) + conj(q2))*sin(q1 + q2 + q3 + q4)*conj(L1)*conj(L2)*sin(q1) + L1*L4*cos(conj(q1) + conj(q2) + conj(q3))*sin(conj(q1) + conj(q2))*sin(q1 + q2 + q3 + q4)*conj(L2)*conj(L3)*sin(q1) - L1*L4*sin(conj(q1) + conj(q2) + conj(q3))*cos(conj(q1) + conj(q2))*sin(q1 + q2 + q3 + q4)*conj(L2)*conj(L3)*sin(q1) + L1*L4*sin(conj(q1) + conj(q2) + conj(q3))*sin(conj(q1) + conj(q2))*cos(q1 + q2 + q3 + q4)*conj(L2)*conj(L3)*sin(q1) - L1*L4*sin(conj(q1) + conj(q2) + conj(q3))*sin(conj(q1) + conj(q2))*sin(q1 + q2 + q3 + q4)*conj(L2)*conj(L3)*cos(q1) + L2*L3*cos(conj(q1) + conj(q2) + conj(q3) + conj(q4))*sin(q1 + q2 + q3)*sin(conj(q1))*conj(L1)*conj(L4)*sin(q1 + q2) + L2*L3*cos(q1 + q2 + q3)*sin(conj(q1) + conj(q2) + conj(q3) + conj(q4))*sin(conj(q1))*conj(L1)*conj(L4)*sin(q1 + q2) - L2*L3*sin(conj(q1) + conj(q2) + conj(q3) + conj(q4))*sin(q1 + q2 + q3)*cos(conj(q1))*conj(L1)*conj(L4)*sin(q1 + q2) - L2*L3*sin(conj(q1) + conj(q2) + conj(q3) + conj(q4))*sin(q1 + q2 + q3)*sin(conj(q1))*cos(q1 + q2)*conj(L1)*conj(L4) + L2*L3*cos(q1 + q2 + q3)*cos(conj(q1))*cos(conj(q1) + conj(q2) + conj(q3))*conj(L1)*conj(L3)*sin(q1 + q2) - L2*L3*cos(q1 + q2 + q3)*cos(conj(q1))*sin(conj(q1) + conj(q2) + conj(q3))*cos(q1 + q2)*conj(L1)*conj(L3) + L2*L3*cos(q1 + q2 + q3)*cos(conj(q1) + conj(q2) + conj(q3))*sin(conj(q1))*cos(q1 + q2)*conj(L1)*conj(L3) - L2*L3*sin(q1 + q2 + q3)*cos(conj(q1))*cos(conj(q1) + conj(q2) + conj(q3))*cos(q1 + q2)*conj(L1)*conj(L3) + 2*L1*L3*cos(conj(q1) + conj(q2) + conj(q3) + conj(q4))*cos(q1 + q2 + q3)*cos(conj(q1))*conj(L1)*conj(L4)*sin(q1) + 2*L1*L3*cos(conj(q1) + conj(q2) + conj(q3) + conj(q4))*cos(q1 + q2 + q3)*sin(conj(q1))*conj(L1)*conj(L4)*cos(q1) - 2*L1*L3*cos(conj(q1) + conj(q2) + conj(q3) + conj(q4))*sin(q1 + q2 + q3)*cos(conj(q1))*conj(L1)*conj(L4)*cos(q1) - 2*L1*L3*cos(q1 + q2 + q3)*sin(conj(q1) + conj(q2) + conj(q3) + conj(q4))*cos(conj(q1))*conj(L1)*conj(L4)*cos(q1) + 2*L2*L3*cos(conj(q1) + conj(q2) + conj(q3) + conj(q4))*cos(q1 + q2 + q3)*cos(conj(q1) + conj(q2))*conj(L2)*conj(L4)*sin(q1 + q2) + 2*L2*L3*cos(conj(q1) + conj(q2) + conj(q3) + conj(q4))*cos(q1 + q2 + q3)*sin(conj(q1) + conj(q2))*cos(q1 + q2)*conj(L2)*conj(L4) - 2*L2*L3*cos(conj(q1) + conj(q2) + conj(q3) + conj(q4))*sin(q1 + q2 + q3)*cos(conj(q1) + conj(q2))*cos(q1 + q2)*conj(L2)*conj(L4) - 2*L2*L3*cos(q1 + q2 + q3)*sin(conj(q1) + conj(q2) + conj(q3) + conj(q4))*cos(conj(q1) + conj(q2))*cos(q1 + q2)*conj(L2)*conj(L4) - 2*L3*L4*cos(q1 + q2 + q3)*sin(conj(q1) + conj(q2) + conj(q3) + conj(q4))*sin(conj(q1) + conj(q2))*sin(q1 + q2 + q3 + q4)*conj(L2)*conj(L4) + 2*L3*L4*sin(conj(q1) + conj(q2) + conj(q3) + conj(q4))*sin(q1 + q2 + q3)*sin(conj(q1) + conj(q2))*cos(q1 + q2 + q3 + q4)*conj(L2)*conj(L4) + L2*L3*cos(q1 + q2 + q3)*sin(conj(q1))*sin(conj(q1) + conj(q2) + conj(q3))*conj(L1)*conj(L3)*sin(q1 + q2) - L2*L3*sin(q1 + q2 + q3)*cos(conj(q1))*sin(conj(q1) + conj(q2) + conj(q3))*conj(L1)*conj(L3)*sin(q1 + q2) + L2*L3*sin(q1 + q2 + q3)*cos(conj(q1) + conj(q2) + conj(q3))*sin(conj(q1))*conj(L1)*conj(L3)*sin(q1 + q2) - L2*L3*sin(q1 + q2 + q3)*sin(conj(q1))*sin(conj(q1) + conj(q2) + conj(q3))*cos(q1 + q2)*conj(L1)*conj(L3) + 2*L1*L3*cos(conj(q1) + conj(q2) + conj(q3) + conj(q4))*sin(q1 + q2 + q3)*sin(conj(q1))*conj(L1)*conj(L4)*sin(q1) + 2*L1*L3*cos(q1 + q2 + q3)*sin(conj(q1) + conj(q2) + conj(q3) + conj(q4))*sin(conj(q1))*conj(L1)*conj(L4)*sin(q1) - 2*L1*L3*sin(conj(q1) + conj(q2) + conj(q3) + conj(q4))*sin(q1 + q2 + q3)*cos(conj(q1))*conj(L1)*conj(L4)*sin(q1) - 2*L1*L3*sin(conj(q1) + conj(q2) + conj(q3) + conj(q4))*sin(q1 + q2 + q3)*sin(conj(q1))*conj(L1)*conj(L4)*cos(q1) + 2*L2*L3*cos(conj(q1) + conj(q2) + conj(q3) + conj(q4))*sin(q1 + q2 + q3)*sin(conj(q1) + conj(q2))*conj(L2)*conj(L4)*sin(q1 + q2) + 2*L2*L3*cos(q1 + q2 + q3)*sin(conj(q1) + conj(q2) + conj(q3) + conj(q4))*sin(conj(q1) + conj(q2))*conj(L2)*conj(L4)*sin(q1 + q2) - 2*L2*L3*sin(conj(q1) + conj(q2) + conj(q3) + conj(q4))*sin(q1 + q2 + q3)*cos(conj(q1) + conj(q2))*conj(L2)*conj(L4)*sin(q1 + q2) - 2*L2*L3*sin(conj(q1) + conj(q2) + conj(q3) + conj(q4))*sin(q1 + q2 + q3)*sin(conj(q1) + conj(q2))*cos(q1 + q2)*conj(L2)*conj(L4) + 2*L1*L3*cos(q1 + q2 + q3)*cos(conj(q1))*cos(conj(q1) + conj(q2) + conj(q3))*conj(L1)*conj(L3)*sin(q1) - 2*L1*L3*cos(q1 + q2 + q3)*cos(conj(q1))*sin(conj(q1) + conj(q2) + conj(q3))*conj(L1)*conj(L3)*cos(q1) + 2*L1*L3*cos(q1 + q2 + q3)*cos(conj(q1) + conj(q2) + conj(q3))*sin(conj(q1))*conj(L1)*conj(L3)*cos(q1) - 2*L1*L3*sin(q1 + q2 + q3)*cos(conj(q1))*cos(conj(q1) + conj(q2) + conj(q3))*conj(L1)*conj(L3)*cos(q1) + 2*L2*L3*cos(q1 + q2 + q3)*cos(conj(q1) + conj(q2) + conj(q3))*cos(conj(q1) + conj(q2))*conj(L2)*conj(L3)*sin(q1 + q2) + 2*L2*L3*cos(q1 + q2 + q3)*cos(conj(q1) + conj(q2) + conj(q3))*sin(conj(q1) + conj(q2))*cos(q1 + q2)*conj(L2)*conj(L3) - 2*L2*L3*cos(q1 + q2 + q3)*sin(conj(q1) + conj(q2) + conj(q3))*cos(conj(q1) + conj(q2))*cos(q1 + q2)*conj(L2)*conj(L3) - 2*L2*L3*sin(q1 + q2 + q3)*cos(conj(q1) + conj(q2) + conj(q3))*cos(conj(q1) + conj(q2))*cos(q1 + q2)*conj(L2)*conj(L3) + L1*L3*cos(conj(q1) + conj(q2) + conj(q3) + conj(q4))*cos(q1 + q2 + q3)*cos(conj(q1) + conj(q2))*conj(L2)*conj(L4)*sin(q1) + L1*L3*cos(conj(q1) + conj(q2) + conj(q3) + conj(q4))*cos(q1 + q2 + q3)*sin(conj(q1) + conj(q2))*conj(L2)*conj(L4)*cos(q1) - L1*L3*cos(conj(q1) + conj(q2) + conj(q3) + conj(q4))*sin(q1 + q2 + q3)*cos(conj(q1) + conj(q2))*conj(L2)*conj(L4)*cos(q1) - L1*L3*cos(q1 + q2 + q3)*sin(conj(q1) + conj(q2) + conj(q3) + conj(q4))*cos(conj(q1) + conj(q2))*conj(L2)*conj(L4)*cos(q1) + 2*L2*L4*cos(conj(q1) + conj(q2) + conj(q3) + conj(q4))*cos(conj(q1))*cos(q1 + q2 + q3 + q4)*conj(L1)*conj(L4)*sin(q1 + q2) - 2*L2*L4*cos(conj(q1) + conj(q2) + conj(q3) + conj(q4))*cos(conj(q1))*sin(q1 + q2 + q3 + q4)*cos(q1 + q2)*conj(L1)*conj(L4) + 2*L2*L4*cos(conj(q1) + conj(q2) + conj(q3) + conj(q4))*sin(conj(q1))*cos(q1 + q2 + q3 + q4)*cos(q1 + q2)*conj(L1)*conj(L4) - 2*L2*L4*sin(conj(q1) + conj(q2) + conj(q3) + conj(q4))*cos(conj(q1))*cos(q1 + q2 + q3 + q4)*cos(q1 + q2)*conj(L1)*conj(L4) + 2*L2*L4*cos(conj(q1) + conj(q2) + conj(q3) + conj(q4))*sin(conj(q1) + conj(q2) + conj(q3))*cos(q1 + q2 + q3 + q4)*cos(q1 + q2)*conj(L3)*conj(L4) - 2*L2*L4*sin(conj(q1) + conj(q2) + conj(q3) + conj(q4))*cos(conj(q1) + conj(q2) + conj(q3))*cos(q1 + q2 + q3 + q4)*cos(q1 + q2)*conj(L3)*conj(L4) + 2*L1*L3*cos(q1 + q2 + q3)*sin(conj(q1))*sin(conj(q1) + conj(q2) + conj(q3))*conj(L1)*conj(L3)*sin(q1) - 2*L1*L3*sin(q1 + q2 + q3)*cos(conj(q1))*sin(conj(q1) + conj(q2) + conj(q3))*conj(L1)*conj(L3)*sin(q1) + 2*L1*L3*sin(q1 + q2 + q3)*cos(conj(q1) + conj(q2) + conj(q3))*sin(conj(q1))*conj(L1)*conj(L3)*sin(q1) - 2*L1*L3*sin(q1 + q2 + q3)*sin(conj(q1))*sin(conj(q1) + conj(q2) + conj(q3))*conj(L1)*conj(L3)*cos(q1) + 2*L2*L3*cos(q1 + q2 + q3)*sin(conj(q1) + conj(q2) + conj(q3))*sin(conj(q1) + conj(q2))*conj(L2)*conj(L3)*sin(q1 + q2) + 2*L2*L3*sin(q1 + q2 + q3)*cos(conj(q1) + conj(q2) + conj(q3))*sin(conj(q1) + conj(q2))*conj(L2)*conj(L3)*sin(q1 + q2) - 2*L2*L3*sin(q1 + q2 + q3)*sin(conj(q1) + conj(q2) + conj(q3))*cos(conj(q1) + conj(q2))*conj(L2)*conj(L3)*sin(q1 + q2) - 2*L2*L3*sin(q1 + q2 + q3)*sin(conj(q1) + conj(q2) + conj(q3))*sin(conj(q1) + conj(q2))*cos(q1 + q2)*conj(L2)*conj(L3) + L1*L3*cos(conj(q1) + conj(q2) + conj(q3) + conj(q4))*sin(q1 + q2 + q3)*sin(conj(q1) + conj(q2))*conj(L2)*conj(L4)*sin(q1) + L1*L3*cos(q1 + q2 + q3)*sin(conj(q1) + conj(q2) + conj(q3) + conj(q4))*sin(conj(q1) + conj(q2))*conj(L2)*conj(L4)*sin(q1) - L1*L3*sin(conj(q1) + conj(q2) + conj(q3) + conj(q4))*sin(q1 + q2 + q3)*cos(conj(q1) + conj(q2))*conj(L2)*conj(L4)*sin(q1) - L1*L3*sin(conj(q1) + conj(q2) + conj(q3) + conj(q4))*sin(q1 + q2 + q3)*sin(conj(q1) + conj(q2))*conj(L2)*conj(L4)*cos(q1) - L1*L3*cos(q1 + q2 + q3)*cos(conj(q1))*sin(conj(q1) + conj(q2))*conj(L1)*conj(L2)*cos(q1) + L1*L3*cos(q1 + q2 + q3)*sin(conj(q1))*cos(conj(q1) + conj(q2))*conj(L1)*conj(L2)*cos(q1) + L1*L3*cos(q1 + q2 + q3)*cos(conj(q1) + conj(q2) + conj(q3))*cos(conj(q1) + conj(q2))*conj(L2)*conj(L3)*sin(q1) + L1*L3*cos(q1 + q2 + q3)*cos(conj(q1) + conj(q2) + conj(q3))*sin(conj(q1) + conj(q2))*conj(L2)*conj(L3)*cos(q1) - L1*L3*cos(q1 + q2 + q3)*sin(conj(q1) + conj(q2) + conj(q3))*cos(conj(q1) + conj(q2))*conj(L2)*conj(L3)*cos(q1) - L1*L3*sin(q1 + q2 + q3)*cos(conj(q1) + conj(q2) + conj(q3))*cos(conj(q1) + conj(q2))*conj(L2)*conj(L3)*cos(q1) + 2*L2*L4*cos(conj(q1) + conj(q2) + conj(q3) + conj(q4))*sin(conj(q1))*sin(q1 + q2 + q3 + q4)*conj(L1)*conj(L4)*sin(q1 + q2) - 2*L2*L4*sin(conj(q1) + conj(q2) + conj(q3) + conj(q4))*cos(conj(q1))*sin(q1 + q2 + q3 + q4)*conj(L1)*conj(L4)*sin(q1 + q2) + 2*L2*L4*sin(conj(q1) + conj(q2) + conj(q3) + conj(q4))*sin(conj(q1))*cos(q1 + q2 + q3 + q4)*conj(L1)*conj(L4)*sin(q1 + q2) - 2*L2*L4*sin(conj(q1) + conj(q2) + conj(q3) + conj(q4))*sin(conj(q1))*sin(q1 + q2 + q3 + q4)*cos(q1 + q2)*conj(L1)*conj(L4)))/(L1*L3*cos(q1 + q2 + q3)*sin(conj(q1))*cos(conj(q1) + conj(q2))*conj(L1)*conj(L2)*sin(q1) - L1*L3*cos(q1 + q2 + q3)*cos(conj(q1))*sin(conj(q1) + conj(q2))*conj(L1)*conj(L2)*sin(q1) + L1*L3*sin(q1 + q2 + q3)*cos(conj(q1))*sin(conj(q1) + conj(q2))*conj(L1)*conj(L2)*cos(q1) - L1*L3*sin(q1 + q2 + q3)*sin(conj(q1))*cos(conj(q1) + conj(q2))*conj(L1)*conj(L2)*cos(q1) + L1*L3*cos(q1 + q2 + q3)*cos(conj(q1) + conj(q2) + conj(q3))*sin(conj(q1) + conj(q2))*conj(L2)*conj(L3)*sin(q1) - L1*L3*cos(q1 + q2 + q3)*sin(conj(q1) + conj(q2) + conj(q3))*cos(conj(q1) + conj(q2))*conj(L2)*conj(L3)*sin(q1) - L1*L3*sin(q1 + q2 + q3)*cos(conj(q1) + conj(q2) + conj(q3))*sin(conj(q1) + conj(q2))*conj(L2)*conj(L3)*cos(q1) + L1*L3*sin(q1 + q2 + q3)*sin(conj(q1) + conj(q2) + conj(q3))*cos(conj(q1) + conj(q2))*conj(L2)*conj(L3)*cos(q1) - L2*L4*cos(conj(q1))*sin(conj(q1) + conj(q2) + conj(q3))*cos(q1 + q2 + q3 + q4)*conj(L1)*conj(L3)*sin(q1 + q2) + L2*L4*cos(conj(q1))*sin(conj(q1) + conj(q2) + conj(q3))*sin(q1 + q2 + q3 + q4)*cos(q1 + q2)*conj(L1)*conj(L3) + L2*L4*cos(conj(q1) + conj(q2) + conj(q3))*sin(conj(q1))*cos(q1 + q2 + q3 + q4)*conj(L1)*conj(L3)*sin(q1 + q2) - L2*L4*cos(conj(q1) + conj(q2) + conj(q3))*sin(conj(q1))*sin(q1 + q2 + q3 + q4)*cos(q1 + q2)*conj(L1)*conj(L3) + 3*L1*L4*cos(conj(q1) + conj(q2) + conj(q3) + conj(q4))*sin(conj(q1))*cos(q1 + q2 + q3 + q4)*conj(L1)*conj(L4)*sin(q1) - 3*L1*L4*cos(conj(q1) + conj(q2) + conj(q3) + conj(q4))*sin(conj(q1))*sin(q1 + q2 + q3 + q4)*conj(L1)*conj(L4)*cos(q1) - 3*L1*L4*sin(conj(q1) + conj(q2) + conj(q3) + conj(q4))*cos(conj(q1))*cos(q1 + q2 + q3 + q4)*conj(L1)*conj(L4)*sin(q1) + 3*L1*L4*sin(conj(q1) + conj(q2) + conj(q3) + conj(q4))*cos(conj(q1))*sin(q1 + q2 + q3 + q4)*conj(L1)*conj(L4)*cos(q1) + 4*L2*L4*cos(conj(q1) + conj(q2) + conj(q3) + conj(q4))*sin(conj(q1) + conj(q2))*cos(q1 + q2 + q3 + q4)*conj(L2)*conj(L4)*sin(q1 + q2) - 4*L2*L4*cos(conj(q1) + conj(q2) + conj(q3) + conj(q4))*sin(conj(q1) + conj(q2))*sin(q1 + q2 + q3 + q4)*cos(q1 + q2)*conj(L2)*conj(L4) - 4*L2*L4*sin(conj(q1) + conj(q2) + conj(q3) + conj(q4))*cos(conj(q1) + conj(q2))*cos(q1 + q2 + q3 + q4)*conj(L2)*conj(L4)*sin(q1 + q2) + 4*L2*L4*sin(conj(q1) + conj(q2) + conj(q3) + conj(q4))*cos(conj(q1) + conj(q2))*sin(q1 + q2 + q3 + q4)*cos(q1 + q2)*conj(L2)*conj(L4) + L1*L4*cos(conj(q1) + conj(q2) + conj(q3) + conj(q4))*sin(conj(q1) + conj(q2) + conj(q3))*cos(q1 + q2 + q3 + q4)*conj(L3)*conj(L4)*sin(q1) - L1*L4*cos(conj(q1) + conj(q2) + conj(q3) + conj(q4))*sin(conj(q1) + conj(q2) + conj(q3))*sin(q1 + q2 + q3 + q4)*conj(L3)*conj(L4)*cos(q1) - L1*L4*sin(conj(q1) + conj(q2) + conj(q3) + conj(q4))*cos(conj(q1) + conj(q2) + conj(q3))*cos(q1 + q2 + q3 + q4)*conj(L3)*conj(L4)*sin(q1) + L1*L4*sin(conj(q1) + conj(q2) + conj(q3) + conj(q4))*cos(conj(q1) + conj(q2) + conj(q3))*sin(q1 + q2 + q3 + q4)*conj(L3)*conj(L4)*cos(q1) + L1*L2*cos(conj(q1) + conj(q2) + conj(q3) + conj(q4))*sin(conj(q1))*cos(q1 + q2)*conj(L1)*conj(L4)*sin(q1) - L1*L2*cos(conj(q1) + conj(q2) + conj(q3) + conj(q4))*sin(conj(q1))*conj(L1)*conj(L4)*sin(q1 + q2)*cos(q1) - L1*L2*sin(conj(q1) + conj(q2) + conj(q3) + conj(q4))*cos(conj(q1))*cos(q1 + q2)*conj(L1)*conj(L4)*sin(q1) + L1*L2*sin(conj(q1) + conj(q2) + conj(q3) + conj(q4))*cos(conj(q1))*conj(L1)*conj(L4)*sin(q1 + q2)*cos(q1) - 2*L1*L4*cos(conj(q1))*sin(conj(q1) + conj(q2) + conj(q3))*cos(q1 + q2 + q3 + q4)*conj(L1)*conj(L3)*sin(q1) + 2*L1*L4*cos(conj(q1))*sin(conj(q1) + conj(q2) + conj(q3))*sin(q1 + q2 + q3 + q4)*conj(L1)*conj(L3)*cos(q1) + 2*L1*L4*cos(conj(q1) + conj(q2) + conj(q3))*sin(conj(q1))*cos(q1 + q2 + q3 + q4)*conj(L1)*conj(L3)*sin(q1) - 2*L1*L4*cos(conj(q1) + conj(q2) + conj(q3))*sin(conj(q1))*sin(q1 + q2 + q3 + q4)*conj(L1)*conj(L3)*cos(q1) + 2*L2*L4*cos(conj(q1) + conj(q2) + conj(q3))*sin(conj(q1) + conj(q2))*cos(q1 + q2 + q3 + q4)*conj(L2)*conj(L3)*sin(q1 + q2) - 2*L2*L4*cos(conj(q1) + conj(q2) + conj(q3))*sin(conj(q1) + conj(q2))*sin(q1 + q2 + q3 + q4)*cos(q1 + q2)*conj(L2)*conj(L3) - 2*L2*L4*sin(conj(q1) + conj(q2) + conj(q3))*cos(conj(q1) + conj(q2))*cos(q1 + q2 + q3 + q4)*conj(L2)*conj(L3)*sin(q1 + q2) + 2*L2*L4*sin(conj(q1) + conj(q2) + conj(q3))*cos(conj(q1) + conj(q2))*sin(q1 + q2 + q3 + q4)*cos(q1 + q2)*conj(L2)*conj(L3) + 2*L1*L4*cos(conj(q1) + conj(q2) + conj(q3) + conj(q4))*sin(conj(q1) + conj(q2))*cos(q1 + q2 + q3 + q4)*conj(L2)*conj(L4)*sin(q1) - 2*L1*L4*cos(conj(q1) + conj(q2) + conj(q3) + conj(q4))*sin(conj(q1) + conj(q2))*sin(q1 + q2 + q3 + q4)*conj(L2)*conj(L4)*cos(q1) - 2*L1*L4*sin(conj(q1) + conj(q2) + conj(q3) + conj(q4))*cos(conj(q1) + conj(q2))*cos(q1 + q2 + q3 + q4)*conj(L2)*conj(L4)*sin(q1) + 2*L1*L4*sin(conj(q1) + conj(q2) + conj(q3) + conj(q4))*cos(conj(q1) + conj(q2))*sin(q1 + q2 + q3 + q4)*conj(L2)*conj(L4)*cos(q1) - L3*L4*cos(conj(q1) + conj(q2) + conj(q3) + conj(q4))*cos(q1 + q2 + q3)*sin(conj(q1))*sin(q1 + q2 + q3 + q4)*conj(L1)*conj(L4) + L3*L4*cos(conj(q1) + conj(q2) + conj(q3) + conj(q4))*sin(q1 + q2 + q3)*sin(conj(q1))*cos(q1 + q2 + q3 + q4)*conj(L1)*conj(L4) + L3*L4*cos(q1 + q2 + q3)*sin(conj(q1) + conj(q2) + conj(q3) + conj(q4))*cos(conj(q1))*sin(q1 + q2 + q3 + q4)*conj(L1)*conj(L4) - L3*L4*sin(conj(q1) + conj(q2) + conj(q3) + conj(q4))*sin(q1 + q2 + q3)*cos(conj(q1))*cos(q1 + q2 + q3 + q4)*conj(L1)*conj(L4) - L1*L2*cos(conj(q1))*sin(conj(q1) + conj(q2) + conj(q3))*cos(q1 + q2)*conj(L1)*conj(L3)*sin(q1) + L1*L2*cos(conj(q1))*sin(conj(q1) + conj(q2) + conj(q3))*conj(L1)*conj(L3)*sin(q1 + q2)*cos(q1) + L1*L2*cos(conj(q1) + conj(q2) + conj(q3))*sin(conj(q1))*cos(q1 + q2)*conj(L1)*conj(L3)*sin(q1) - L1*L2*cos(conj(q1) + conj(q2) + conj(q3))*sin(conj(q1))*conj(L1)*conj(L3)*sin(q1 + q2)*cos(q1) - 3*L3*L4*cos(conj(q1) + conj(q2) + conj(q3) + conj(q4))*cos(q1 + q2 + q3)*sin(conj(q1) + conj(q2) + conj(q3))*sin(q1 + q2 + q3 + q4)*conj(L3)*conj(L4) + 3*L3*L4*cos(conj(q1) + conj(q2) + conj(q3) + conj(q4))*sin(q1 + q2 + q3)*sin(conj(q1) + conj(q2) + conj(q3))*cos(q1 + q2 + q3 + q4)*conj(L3)*conj(L4) + 3*L3*L4*cos(q1 + q2 + q3)*sin(conj(q1) + conj(q2) + conj(q3) + conj(q4))*cos(conj(q1) + conj(q2) + conj(q3))*sin(q1 + q2 + q3 + q4)*conj(L3)*conj(L4) - 3*L3*L4*sin(conj(q1) + conj(q2) + conj(q3) + conj(q4))*sin(q1 + q2 + q3)*cos(conj(q1) + conj(q2) + conj(q3))*cos(q1 + q2 + q3 + q4)*conj(L3)*conj(L4) - L1*L4*cos(conj(q1))*sin(conj(q1) + conj(q2))*cos(q1 + q2 + q3 + q4)*conj(L1)*conj(L2)*sin(q1) + L1*L4*cos(conj(q1))*sin(conj(q1) + conj(q2))*sin(q1 + q2 + q3 + q4)*conj(L1)*conj(L2)*cos(q1) + L1*L4*sin(conj(q1))*cos(conj(q1) + conj(q2))*cos(q1 + q2 + q3 + q4)*conj(L1)*conj(L2)*sin(q1) - L1*L4*sin(conj(q1))*cos(conj(q1) + conj(q2))*sin(q1 + q2 + q3 + q4)*conj(L1)*conj(L2)*cos(q1) + L1*L4*cos(conj(q1) + conj(q2) + conj(q3))*sin(conj(q1) + conj(q2))*cos(q1 + q2 + q3 + q4)*conj(L2)*conj(L3)*sin(q1) - L1*L4*cos(conj(q1) + conj(q2) + conj(q3))*sin(conj(q1) + conj(q2))*sin(q1 + q2 + q3 + q4)*conj(L2)*conj(L3)*cos(q1) - L1*L4*sin(conj(q1) + conj(q2) + conj(q3))*cos(conj(q1) + conj(q2))*cos(q1 + q2 + q3 + q4)*conj(L2)*conj(L3)*sin(q1) + L1*L4*sin(conj(q1) + conj(q2) + conj(q3))*cos(conj(q1) + conj(q2))*sin(q1 + q2 + q3 + q4)*conj(L2)*conj(L3)*cos(q1) + L2*L3*cos(conj(q1) + conj(q2) + conj(q3) + conj(q4))*cos(q1 + q2 + q3)*sin(conj(q1))*conj(L1)*conj(L4)*sin(q1 + q2) - L2*L3*cos(conj(q1) + conj(q2) + conj(q3) + conj(q4))*sin(q1 + q2 + q3)*sin(conj(q1))*cos(q1 + q2)*conj(L1)*conj(L4) - L2*L3*cos(q1 + q2 + q3)*sin(conj(q1) + conj(q2) + conj(q3) + conj(q4))*cos(conj(q1))*conj(L1)*conj(L4)*sin(q1 + q2) + L2*L3*sin(conj(q1) + conj(q2) + conj(q3) + conj(q4))*sin(q1 + q2 + q3)*cos(conj(q1))*cos(q1 + q2)*conj(L1)*conj(L4) - L1*L2*cos(conj(q1))*sin(conj(q1) + conj(q2))*cos(q1 + q2)*conj(L1)*conj(L2)*sin(q1) + L1*L2*cos(conj(q1))*sin(conj(q1) + conj(q2))*conj(L1)*conj(L2)*sin(q1 + q2)*cos(q1) + L1*L2*sin(conj(q1))*cos(conj(q1) + conj(q2))*cos(q1 + q2)*conj(L1)*conj(L2)*sin(q1) - L1*L2*sin(conj(q1))*cos(conj(q1) + conj(q2))*conj(L1)*conj(L2)*sin(q1 + q2)*cos(q1) - 2*L3*L4*cos(conj(q1) + conj(q2) + conj(q3) + conj(q4))*cos(q1 + q2 + q3)*sin(conj(q1) + conj(q2))*sin(q1 + q2 + q3 + q4)*conj(L2)*conj(L4) + 2*L3*L4*cos(conj(q1) + conj(q2) + conj(q3) + conj(q4))*sin(q1 + q2 + q3)*sin(conj(q1) + conj(q2))*cos(q1 + q2 + q3 + q4)*conj(L2)*conj(L4) + 2*L3*L4*cos(q1 + q2 + q3)*sin(conj(q1) + conj(q2) + conj(q3) + conj(q4))*cos(conj(q1) + conj(q2))*sin(q1 + q2 + q3 + q4)*conj(L2)*conj(L4) - 2*L3*L4*sin(conj(q1) + conj(q2) + conj(q3) + conj(q4))*sin(q1 + q2 + q3)*cos(conj(q1) + conj(q2))*cos(q1 + q2 + q3 + q4)*conj(L2)*conj(L4) - L2*L3*cos(q1 + q2 + q3)*cos(conj(q1))*sin(conj(q1) + conj(q2) + conj(q3))*conj(L1)*conj(L3)*sin(q1 + q2) + L2*L3*cos(q1 + q2 + q3)*cos(conj(q1) + conj(q2) + conj(q3))*sin(conj(q1))*conj(L1)*conj(L3)*sin(q1 + q2) + L2*L3*sin(q1 + q2 + q3)*cos(conj(q1))*sin(conj(q1) + conj(q2) + conj(q3))*cos(q1 + q2)*conj(L1)*conj(L3) - L2*L3*sin(q1 + q2 + q3)*cos(conj(q1) + conj(q2) + conj(q3))*sin(conj(q1))*cos(q1 + q2)*conj(L1)*conj(L3) + 2*L1*L3*cos(conj(q1) + conj(q2) + conj(q3) + conj(q4))*cos(q1 + q2 + q3)*sin(conj(q1))*conj(L1)*conj(L4)*sin(q1) - 2*L1*L3*cos(conj(q1) + conj(q2) + conj(q3) + conj(q4))*sin(q1 + q2 + q3)*sin(conj(q1))*conj(L1)*conj(L4)*cos(q1) - 2*L1*L3*cos(q1 + q2 + q3)*sin(conj(q1) + conj(q2) + conj(q3) + conj(q4))*cos(conj(q1))*conj(L1)*conj(L4)*sin(q1) + 2*L1*L3*sin(conj(q1) + conj(q2) + conj(q3) + conj(q4))*sin(q1 + q2 + q3)*cos(conj(q1))*conj(L1)*conj(L4)*cos(q1) + 2*L2*L3*cos(conj(q1) + conj(q2) + conj(q3) + conj(q4))*cos(q1 + q2 + q3)*sin(conj(q1) + conj(q2))*conj(L2)*conj(L4)*sin(q1 + q2) - 2*L2*L3*cos(conj(q1) + conj(q2) + conj(q3) + conj(q4))*sin(q1 + q2 + q3)*sin(conj(q1) + conj(q2))*cos(q1 + q2)*conj(L2)*conj(L4) - 2*L2*L3*cos(q1 + q2 + q3)*sin(conj(q1) + conj(q2) + conj(q3) + conj(q4))*cos(conj(q1) + conj(q2))*conj(L2)*conj(L4)*sin(q1 + q2) + 2*L2*L3*sin(conj(q1) + conj(q2) + conj(q3) + conj(q4))*sin(q1 + q2 + q3)*cos(conj(q1) + conj(q2))*cos(q1 + q2)*conj(L2)*conj(L4) - 2*L1*L3*cos(q1 + q2 + q3)*cos(conj(q1))*sin(conj(q1) + conj(q2) + conj(q3))*conj(L1)*conj(L3)*sin(q1) + 2*L1*L3*cos(q1 + q2 + q3)*cos(conj(q1) + conj(q2) + conj(q3))*sin(conj(q1))*conj(L1)*conj(L3)*sin(q1) + 2*L1*L3*sin(q1 + q2 + q3)*cos(conj(q1))*sin(conj(q1) + conj(q2) + conj(q3))*conj(L1)*conj(L3)*cos(q1) - 2*L1*L3*sin(q1 + q2 + q3)*cos(conj(q1) + conj(q2) + conj(q3))*sin(conj(q1))*conj(L1)*conj(L3)*cos(q1) + 2*L2*L3*cos(q1 + q2 + q3)*cos(conj(q1) + conj(q2) + conj(q3))*sin(conj(q1) + conj(q2))*conj(L2)*conj(L3)*sin(q1 + q2) - 2*L2*L3*cos(q1 + q2 + q3)*sin(conj(q1) + conj(q2) + conj(q3))*cos(conj(q1) + conj(q2))*conj(L2)*conj(L3)*sin(q1 + q2) - 2*L2*L3*sin(q1 + q2 + q3)*cos(conj(q1) + conj(q2) + conj(q3))*sin(conj(q1) + conj(q2))*cos(q1 + q2)*conj(L2)*conj(L3) + 2*L2*L3*sin(q1 + q2 + q3)*sin(conj(q1) + conj(q2) + conj(q3))*cos(conj(q1) + conj(q2))*cos(q1 + q2)*conj(L2)*conj(L3) + L1*L3*cos(conj(q1) + conj(q2) + conj(q3) + conj(q4))*cos(q1 + q2 + q3)*sin(conj(q1) + conj(q2))*conj(L2)*conj(L4)*sin(q1) - L1*L3*cos(conj(q1) + conj(q2) + conj(q3) + conj(q4))*sin(q1 + q2 + q3)*sin(conj(q1) + conj(q2))*conj(L2)*conj(L4)*cos(q1) - L1*L3*cos(q1 + q2 + q3)*sin(conj(q1) + conj(q2) + conj(q3) + conj(q4))*cos(conj(q1) + conj(q2))*conj(L2)*conj(L4)*sin(q1) + L1*L3*sin(conj(q1) + conj(q2) + conj(q3) + conj(q4))*sin(q1 + q2 + q3)*cos(conj(q1) + conj(q2))*conj(L2)*conj(L4)*cos(q1) + 2*L2*L4*cos(conj(q1) + conj(q2) + conj(q3) + conj(q4))*sin(conj(q1))*cos(q1 + q2 + q3 + q4)*conj(L1)*conj(L4)*sin(q1 + q2) - 2*L2*L4*cos(conj(q1) + conj(q2) + conj(q3) + conj(q4))*sin(conj(q1))*sin(q1 + q2 + q3 + q4)*cos(q1 + q2)*conj(L1)*conj(L4) - 2*L2*L4*sin(conj(q1) + conj(q2) + conj(q3) + conj(q4))*cos(conj(q1))*cos(q1 + q2 + q3 + q4)*conj(L1)*conj(L4)*sin(q1 + q2) + 2*L2*L4*sin(conj(q1) + conj(q2) + conj(q3) + conj(q4))*cos(conj(q1))*sin(q1 + q2 + q3 + q4)*cos(q1 + q2)*conj(L1)*conj(L4) + 2*L2*L4*cos(conj(q1) + conj(q2) + conj(q3) + conj(q4))*sin(conj(q1) + conj(q2) + conj(q3))*cos(q1 + q2 + q3 + q4)*conj(L3)*conj(L4)*sin(q1 + q2) - 2*L2*L4*cos(conj(q1) + conj(q2) + conj(q3) + conj(q4))*sin(conj(q1) + conj(q2) + conj(q3))*sin(q1 + q2 + q3 + q4)*cos(q1 + q2)*conj(L3)*conj(L4) - 2*L2*L4*sin(conj(q1) + conj(q2) + conj(q3) + conj(q4))*cos(conj(q1) + conj(q2) + conj(q3))*cos(q1 + q2 + q3 + q4)*conj(L3)*conj(L4)*sin(q1 + q2) + 2*L2*L4*sin(conj(q1) + conj(q2) + conj(q3) + conj(q4))*cos(conj(q1) + conj(q2) + conj(q3))*sin(q1 + q2 + q3 + q4)*cos(q1 + q2)*conj(L3)*conj(L4))^0.5000;
aux41 = (0.5000*(2*L2*L4*cos(conj(q1) + conj(q2) + conj(q3) + conj(q4))*sin(conj(q1) + conj(q2) + conj(q3))*sin(q1 + q2 + q3 + q4)*conj(L3)*conj(L4)*sin(q1 + q2) - 2*L2*L4*sin(conj(q1) + conj(q2) + conj(q3) + conj(q4))*cos(conj(q1) + conj(q2) + conj(q3))*sin(q1 + q2 + q3 + q4)*conj(L3)*conj(L4)*sin(q1 + q2) + 2*L2*L4*sin(conj(q1) + conj(q2) + conj(q3) + conj(q4))*sin(conj(q1) + conj(q2) + conj(q3))*cos(q1 + q2 + q3 + q4)*conj(L3)*conj(L4)*sin(q1 + q2) - 2*L2*L4*sin(conj(q1) + conj(q2) + conj(q3) + conj(q4))*sin(conj(q1) + conj(q2) + conj(q3))*sin(q1 + q2 + q3 + q4)*cos(q1 + q2)*conj(L3)*conj(L4) - L2*L4*cos(conj(q1))*sin(conj(q1) + conj(q2) + conj(q3))*cos(q1 + q2 + q3 + q4)*cos(q1 + q2)*conj(L1)*conj(L3) + L2*L4*cos(conj(q1) + conj(q2) + conj(q3))*sin(conj(q1))*cos(q1 + q2 + q3 + q4)*cos(q1 + q2)*conj(L1)*conj(L3) + 3*L1*L4*cos(conj(q1) + conj(q2) + conj(q3) + conj(q4))*cos(conj(q1))*cos(q1 + q2 + q3 + q4)*conj(L1)*conj(L4)*sin(q1) - 3*L1*L4*cos(conj(q1) + conj(q2) + conj(q3) + conj(q4))*cos(conj(q1))*sin(q1 + q2 + q3 + q4)*conj(L1)*conj(L4)*cos(q1) + 3*L1*L4*cos(conj(q1) + conj(q2) + conj(q3) + conj(q4))*sin(conj(q1))*cos(q1 + q2 + q3 + q4)*conj(L1)*conj(L4)*cos(q1) - 3*L1*L4*sin(conj(q1) + conj(q2) + conj(q3) + conj(q4))*cos(conj(q1))*cos(q1 + q2 + q3 + q4)*conj(L1)*conj(L4)*cos(q1) + 4*L2*L4*cos(conj(q1) + conj(q2) + conj(q3) + conj(q4))*cos(conj(q1) + conj(q2))*cos(q1 + q2 + q3 + q4)*conj(L2)*conj(L4)*sin(q1 + q2) - 4*L2*L4*cos(conj(q1) + conj(q2) + conj(q3) + conj(q4))*cos(conj(q1) + conj(q2))*sin(q1 + q2 + q3 + q4)*cos(q1 + q2)*conj(L2)*conj(L4) + 4*L2*L4*cos(conj(q1) + conj(q2) + conj(q3) + conj(q4))*sin(conj(q1) + conj(q2))*cos(q1 + q2 + q3 + q4)*cos(q1 + q2)*conj(L2)*conj(L4) - 4*L2*L4*sin(conj(q1) + conj(q2) + conj(q3) + conj(q4))*cos(conj(q1) + conj(q2))*cos(q1 + q2 + q3 + q4)*cos(q1 + q2)*conj(L2)*conj(L4) + L1*L4*cos(conj(q1) + conj(q2) + conj(q3) + conj(q4))*cos(conj(q1) + conj(q2) + conj(q3))*cos(q1 + q2 + q3 + q4)*conj(L3)*conj(L4)*sin(q1) - L1*L4*cos(conj(q1) + conj(q2) + conj(q3) + conj(q4))*cos(conj(q1) + conj(q2) + conj(q3))*sin(q1 + q2 + q3 + q4)*conj(L3)*conj(L4)*cos(q1) + L1*L4*cos(conj(q1) + conj(q2) + conj(q3) + conj(q4))*sin(conj(q1) + conj(q2) + conj(q3))*cos(q1 + q2 + q3 + q4)*conj(L3)*conj(L4)*cos(q1) - L1*L4*sin(conj(q1) + conj(q2) + conj(q3) + conj(q4))*cos(conj(q1) + conj(q2) + conj(q3))*cos(q1 + q2 + q3 + q4)*conj(L3)*conj(L4)*cos(q1) - L2*L4*cos(conj(q1))*sin(conj(q1) + conj(q2) + conj(q3))*sin(q1 + q2 + q3 + q4)*conj(L1)*conj(L3)*sin(q1 + q2) + L2*L4*cos(conj(q1) + conj(q2) + conj(q3))*sin(conj(q1))*sin(q1 + q2 + q3 + q4)*conj(L1)*conj(L3)*sin(q1 + q2) + L1*L2*cos(conj(q1) + conj(q2) + conj(q3) + conj(q4))*cos(conj(q1))*cos(q1 + q2)*conj(L1)*conj(L4)*sin(q1) - L1*L2*cos(conj(q1) + conj(q2) + conj(q3) + conj(q4))*cos(conj(q1))*conj(L1)*conj(L4)*sin(q1 + q2)*cos(q1) + 3*L1*L4*cos(conj(q1) + conj(q2) + conj(q3) + conj(q4))*sin(conj(q1))*sin(q1 + q2 + q3 + q4)*conj(L1)*conj(L4)*sin(q1) - 3*L1*L4*sin(conj(q1) + conj(q2) + conj(q3) + conj(q4))*cos(conj(q1))*sin(q1 + q2 + q3 + q4)*conj(L1)*conj(L4)*sin(q1) + 3*L1*L4*sin(conj(q1) + conj(q2) + conj(q3) + conj(q4))*sin(conj(q1))*cos(q1 + q2 + q3 + q4)*conj(L1)*conj(L4)*sin(q1) - 3*L1*L4*sin(conj(q1) + conj(q2) + conj(q3) + conj(q4))*sin(conj(q1))*sin(q1 + q2 + q3 + q4)*conj(L1)*conj(L4)*cos(q1) + 4*L2*L4*cos(conj(q1) + conj(q2) + conj(q3) + conj(q4))*sin(conj(q1) + conj(q2))*sin(q1 + q2 + q3 + q4)*conj(L2)*conj(L4)*sin(q1 + q2) - 4*L2*L4*sin(conj(q1) + conj(q2) + conj(q3) + conj(q4))*cos(conj(q1) + conj(q2))*sin(q1 + q2 + q3 + q4)*conj(L2)*conj(L4)*sin(q1 + q2) + 4*L2*L4*sin(conj(q1) + conj(q2) + conj(q3) + conj(q4))*sin(conj(q1) + conj(q2))*cos(q1 + q2 + q3 + q4)*conj(L2)*conj(L4)*sin(q1 + q2) - 4*L2*L4*sin(conj(q1) + conj(q2) + conj(q3) + conj(q4))*sin(conj(q1) + conj(q2))*sin(q1 + q2 + q3 + q4)*cos(q1 + q2)*conj(L2)*conj(L4) + L1*L4*cos(conj(q1) + conj(q2) + conj(q3) + conj(q4))*sin(conj(q1) + conj(q2) + conj(q3))*sin(q1 + q2 + q3 + q4)*conj(L3)*conj(L4)*sin(q1) - L1*L4*sin(conj(q1) + conj(q2) + conj(q3) + conj(q4))*cos(conj(q1) + conj(q2) + conj(q3))*sin(q1 + q2 + q3 + q4)*conj(L3)*conj(L4)*sin(q1) + L1*L4*sin(conj(q1) + conj(q2) + conj(q3) + conj(q4))*sin(conj(q1) + conj(q2) + conj(q3))*cos(q1 + q2 + q3 + q4)*conj(L3)*conj(L4)*sin(q1) - L1*L4*sin(conj(q1) + conj(q2) + conj(q3) + conj(q4))*sin(conj(q1) + conj(q2) + conj(q3))*sin(q1 + q2 + q3 + q4)*conj(L3)*conj(L4)*cos(q1) - 2*L1*L4*cos(conj(q1))*sin(conj(q1) + conj(q2) + conj(q3))*cos(q1 + q2 + q3 + q4)*conj(L1)*conj(L3)*cos(q1) + 2*L1*L4*cos(conj(q1) + conj(q2) + conj(q3))*sin(conj(q1))*cos(q1 + q2 + q3 + q4)*conj(L1)*conj(L3)*cos(q1) + 2*L2*L4*cos(conj(q1) + conj(q2) + conj(q3))*sin(conj(q1) + conj(q2))*cos(q1 + q2 + q3 + q4)*cos(q1 + q2)*conj(L2)*conj(L3) - 2*L2*L4*sin(conj(q1) + conj(q2) + conj(q3))*cos(conj(q1) + conj(q2))*cos(q1 + q2 + q3 + q4)*cos(q1 + q2)*conj(L2)*conj(L3) + 2*L1*L4*cos(conj(q1) + conj(q2) + conj(q3) + conj(q4))*cos(conj(q1) + conj(q2))*cos(q1 + q2 + q3 + q4)*conj(L2)*conj(L4)*sin(q1) - 2*L1*L4*cos(conj(q1) + conj(q2) + conj(q3) + conj(q4))*cos(conj(q1) + conj(q2))*sin(q1 + q2 + q3 + q4)*conj(L2)*conj(L4)*cos(q1) + 2*L1*L4*cos(conj(q1) + conj(q2) + conj(q3) + conj(q4))*sin(conj(q1) + conj(q2))*cos(q1 + q2 + q3 + q4)*conj(L2)*conj(L4)*cos(q1) - 2*L1*L4*sin(conj(q1) + conj(q2) + conj(q3) + conj(q4))*cos(conj(q1) + conj(q2))*cos(q1 + q2 + q3 + q4)*conj(L2)*conj(L4)*cos(q1) + L1*L2*sin(conj(q1) + conj(q2) + conj(q3) + conj(q4))*sin(conj(q1))*cos(q1 + q2)*conj(L1)*conj(L4)*sin(q1) - L1*L2*sin(conj(q1) + conj(q2) + conj(q3) + conj(q4))*sin(conj(q1))*conj(L1)*conj(L4)*sin(q1 + q2)*cos(q1) - L3*L4*cos(conj(q1) + conj(q2) + conj(q3) + conj(q4))*cos(q1 + q2 + q3)*cos(conj(q1))*sin(q1 + q2 + q3 + q4)*conj(L1)*conj(L4) + L3*L4*cos(conj(q1) + conj(q2) + conj(q3) + conj(q4))*cos(q1 + q2 + q3)*sin(conj(q1))*cos(q1 + q2 + q3 + q4)*conj(L1)*conj(L4) + L3*L4*cos(conj(q1) + conj(q2) + conj(q3) + conj(q4))*sin(q1 + q2 + q3)*cos(conj(q1))*cos(q1 + q2 + q3 + q4)*conj(L1)*conj(L4) - L3*L4*cos(q1 + q2 + q3)*sin(conj(q1) + conj(q2) + conj(q3) + conj(q4))*cos(conj(q1))*cos(q1 + q2 + q3 + q4)*conj(L1)*conj(L4) - 3*L3*L4*cos(conj(q1) + conj(q2) + conj(q3) + conj(q4))*cos(q1 + q2 + q3)*cos(conj(q1) + conj(q2) + conj(q3))*sin(q1 + q2 + q3 + q4)*conj(L3)*conj(L4) + 3*L3*L4*cos(conj(q1) + conj(q2) + conj(q3) + conj(q4))*cos(q1 + q2 + q3)*sin(conj(q1) + conj(q2) + conj(q3))*cos(q1 + q2 + q3 + q4)*conj(L3)*conj(L4) + 3*L3*L4*cos(conj(q1) + conj(q2) + conj(q3) + conj(q4))*sin(q1 + q2 + q3)*cos(conj(q1) + conj(q2) + conj(q3))*cos(q1 + q2 + q3 + q4)*conj(L3)*conj(L4) - 3*L3*L4*cos(q1 + q2 + q3)*sin(conj(q1) + conj(q2) + conj(q3) + conj(q4))*cos(conj(q1) + conj(q2) + conj(q3))*cos(q1 + q2 + q3 + q4)*conj(L3)*conj(L4) - 2*L1*L4*cos(conj(q1))*sin(conj(q1) + conj(q2) + conj(q3))*sin(q1 + q2 + q3 + q4)*conj(L1)*conj(L3)*sin(q1) + 2*L1*L4*cos(conj(q1) + conj(q2) + conj(q3))*sin(conj(q1))*sin(q1 + q2 + q3 + q4)*conj(L1)*conj(L3)*sin(q1) + 2*L2*L4*cos(conj(q1) + conj(q2) + conj(q3))*sin(conj(q1) + conj(q2))*sin(q1 + q2 + q3 + q4)*conj(L2)*conj(L3)*sin(q1 + q2) - 2*L2*L4*sin(conj(q1) + conj(q2) + conj(q3))*cos(conj(q1) + conj(q2))*sin(q1 + q2 + q3 + q4)*conj(L2)*conj(L3)*sin(q1 + q2) + 2*L1*L4*cos(conj(q1) + conj(q2) + conj(q3) + conj(q4))*sin(conj(q1) + conj(q2))*sin(q1 + q2 + q3 + q4)*conj(L2)*conj(L4)*sin(q1) - 2*L1*L4*sin(conj(q1) + conj(q2) + conj(q3) + conj(q4))*cos(conj(q1) + conj(q2))*sin(q1 + q2 + q3 + q4)*conj(L2)*conj(L4)*sin(q1) + 2*L1*L4*sin(conj(q1) + conj(q2) + conj(q3) + conj(q4))*sin(conj(q1) + conj(q2))*cos(q1 + q2 + q3 + q4)*conj(L2)*conj(L4)*sin(q1) - 2*L1*L4*sin(conj(q1) + conj(q2) + conj(q3) + conj(q4))*sin(conj(q1) + conj(q2))*sin(q1 + q2 + q3 + q4)*conj(L2)*conj(L4)*cos(q1) - L1*L4*cos(conj(q1))*sin(conj(q1) + conj(q2))*cos(q1 + q2 + q3 + q4)*conj(L1)*conj(L2)*cos(q1) + L1*L4*sin(conj(q1))*cos(conj(q1) + conj(q2))*cos(q1 + q2 + q3 + q4)*conj(L1)*conj(L2)*cos(q1) + L1*L4*cos(conj(q1) + conj(q2) + conj(q3))*sin(conj(q1) + conj(q2))*cos(q1 + q2 + q3 + q4)*conj(L2)*conj(L3)*cos(q1) - L1*L4*sin(conj(q1) + conj(q2) + conj(q3))*cos(conj(q1) + conj(q2))*cos(q1 + q2 + q3 + q4)*conj(L2)*conj(L3)*cos(q1) + L2*L3*cos(conj(q1) + conj(q2) + conj(q3) + conj(q4))*cos(q1 + q2 + q3)*cos(conj(q1))*conj(L1)*conj(L4)*sin(q1 + q2) - L2*L3*cos(conj(q1) + conj(q2) + conj(q3) + conj(q4))*sin(q1 + q2 + q3)*cos(conj(q1))*cos(q1 + q2)*conj(L1)*conj(L4) + L3*L4*cos(conj(q1) + conj(q2) + conj(q3) + conj(q4))*sin(q1 + q2 + q3)*sin(conj(q1))*sin(q1 + q2 + q3 + q4)*conj(L1)*conj(L4) - L3*L4*cos(q1 + q2 + q3)*sin(conj(q1) + conj(q2) + conj(q3) + conj(q4))*sin(conj(q1))*sin(q1 + q2 + q3 + q4)*conj(L1)*conj(L4) - L3*L4*sin(conj(q1) + conj(q2) + conj(q3) + conj(q4))*sin(q1 + q2 + q3)*cos(conj(q1))*sin(q1 + q2 + q3 + q4)*conj(L1)*conj(L4) + L3*L4*sin(conj(q1) + conj(q2) + conj(q3) + conj(q4))*sin(q1 + q2 + q3)*sin(conj(q1))*cos(q1 + q2 + q3 + q4)*conj(L1)*conj(L4) + 3*L3*L4*cos(conj(q1) + conj(q2) + conj(q3) + conj(q4))*sin(q1 + q2 + q3)*sin(conj(q1) + conj(q2) + conj(q3))*sin(q1 + q2 + q3 + q4)*conj(L3)*conj(L4) - 3*L3*L4*cos(q1 + q2 + q3)*sin(conj(q1) + conj(q2) + conj(q3) + conj(q4))*sin(conj(q1) + conj(q2) + conj(q3))*sin(q1 + q2 + q3 + q4)*conj(L3)*conj(L4) - 3*L3*L4*sin(conj(q1) + conj(q2) + conj(q3) + conj(q4))*sin(q1 + q2 + q3)*cos(conj(q1) + conj(q2) + conj(q3))*sin(q1 + q2 + q3 + q4)*conj(L3)*conj(L4) + 3*L3*L4*sin(conj(q1) + conj(q2) + conj(q3) + conj(q4))*sin(q1 + q2 + q3)*sin(conj(q1) + conj(q2) + conj(q3))*cos(q1 + q2 + q3 + q4)*conj(L3)*conj(L4) - 2*L3*L4*cos(conj(q1) + conj(q2) + conj(q3) + conj(q4))*cos(q1 + q2 + q3)*cos(conj(q1) + conj(q2))*sin(q1 + q2 + q3 + q4)*conj(L2)*conj(L4) + 2*L3*L4*cos(conj(q1) + conj(q2) + conj(q3) + conj(q4))*cos(q1 + q2 + q3)*sin(conj(q1) + conj(q2))*cos(q1 + q2 + q3 + q4)*conj(L2)*conj(L4) + 2*L3*L4*cos(conj(q1) + conj(q2) + conj(q3) + conj(q4))*sin(q1 + q2 + q3)*cos(conj(q1) + conj(q2))*cos(q1 + q2 + q3 + q4)*conj(L2)*conj(L4) - 2*L3*L4*cos(q1 + q2 + q3)*sin(conj(q1) + conj(q2) + conj(q3) + conj(q4))*cos(conj(q1) + conj(q2))*cos(q1 + q2 + q3 + q4)*conj(L2)*conj(L4) - L1*L4*cos(conj(q1))*sin(conj(q1) + conj(q2))*sin(q1 + q2 + q3 + q4)*conj(L1)*conj(L2)*sin(q1) + L1*L4*sin(conj(q1))*cos(conj(q1) + conj(q2))*sin(q1 + q2 + q3 + q4)*conj(L1)*conj(L2)*sin(q1) + L1*L4*cos(conj(q1) + conj(q2) + conj(q3))*sin(conj(q1) + conj(q2))*sin(q1 + q2 + q3 + q4)*conj(L2)*conj(L3)*sin(q1) - L1*L4*sin(conj(q1) + conj(q2) + conj(q3))*cos(conj(q1) + conj(q2))*sin(q1 + q2 + q3 + q4)*conj(L2)*conj(L3)*sin(q1) + L2*L3*cos(q1 + q2 + q3)*sin(conj(q1) + conj(q2) + conj(q3) + conj(q4))*sin(conj(q1))*conj(L1)*conj(L4)*sin(q1 + q2) - L2*L3*sin(conj(q1) + conj(q2) + conj(q3) + conj(q4))*sin(q1 + q2 + q3)*sin(conj(q1))*cos(q1 + q2)*conj(L1)*conj(L4) + 2*L1*L3*cos(conj(q1) + conj(q2) + conj(q3) + conj(q4))*cos(q1 + q2 + q3)*cos(conj(q1))*conj(L1)*conj(L4)*sin(q1) - 2*L1*L3*cos(conj(q1) + conj(q2) + conj(q3) + conj(q4))*sin(q1 + q2 + q3)*cos(conj(q1))*conj(L1)*conj(L4)*cos(q1) + 2*L2*L3*cos(conj(q1) + conj(q2) + conj(q3) + conj(q4))*cos(q1 + q2 + q3)*cos(conj(q1) + conj(q2))*conj(L2)*conj(L4)*sin(q1 + q2) - 2*L2*L3*cos(conj(q1) + conj(q2) + conj(q3) + conj(q4))*sin(q1 + q2 + q3)*cos(conj(q1) + conj(q2))*cos(q1 + q2)*conj(L2)*conj(L4) + 2*L3*L4*cos(conj(q1) + conj(q2) + conj(q3) + conj(q4))*sin(q1 + q2 + q3)*sin(conj(q1) + conj(q2))*sin(q1 + q2 + q3 + q4)*conj(L2)*conj(L4) - 2*L3*L4*cos(q1 + q2 + q3)*sin(conj(q1) + conj(q2) + conj(q3) + conj(q4))*sin(conj(q1) + conj(q2))*sin(q1 + q2 + q3 + q4)*conj(L2)*conj(L4) - 2*L3*L4*sin(conj(q1) + conj(q2) + conj(q3) + conj(q4))*sin(q1 + q2 + q3)*cos(conj(q1) + conj(q2))*sin(q1 + q2 + q3 + q4)*conj(L2)*conj(L4) + 2*L3*L4*sin(conj(q1) + conj(q2) + conj(q3) + conj(q4))*sin(q1 + q2 + q3)*sin(conj(q1) + conj(q2))*cos(q1 + q2 + q3 + q4)*conj(L2)*conj(L4) + 2*L1*L3*cos(q1 + q2 + q3)*sin(conj(q1) + conj(q2) + conj(q3) + conj(q4))*sin(conj(q1))*conj(L1)*conj(L4)*sin(q1) - 2*L1*L3*sin(conj(q1) + conj(q2) + conj(q3) + conj(q4))*sin(q1 + q2 + q3)*sin(conj(q1))*conj(L1)*conj(L4)*cos(q1) + 2*L2*L3*cos(q1 + q2 + q3)*sin(conj(q1) + conj(q2) + conj(q3) + conj(q4))*sin(conj(q1) + conj(q2))*conj(L2)*conj(L4)*sin(q1 + q2) - 2*L2*L3*sin(conj(q1) + conj(q2) + conj(q3) + conj(q4))*sin(q1 + q2 + q3)*sin(conj(q1) + conj(q2))*cos(q1 + q2)*conj(L2)*conj(L4) + L1*L3*cos(conj(q1) + conj(q2) + conj(q3) + conj(q4))*cos(q1 + q2 + q3)*cos(conj(q1) + conj(q2))*conj(L2)*conj(L4)*sin(q1) - L1*L3*cos(conj(q1) + conj(q2) + conj(q3) + conj(q4))*sin(q1 + q2 + q3)*cos(conj(q1) + conj(q2))*conj(L2)*conj(L4)*cos(q1) + 2*L2*L4*cos(conj(q1) + conj(q2) + conj(q3) + conj(q4))*cos(conj(q1))*cos(q1 + q2 + q3 + q4)*conj(L1)*conj(L4)*sin(q1 + q2) - 2*L2*L4*cos(conj(q1) + conj(q2) + conj(q3) + conj(q4))*cos(conj(q1))*sin(q1 + q2 + q3 + q4)*cos(q1 + q2)*conj(L1)*conj(L4) + 2*L2*L4*cos(conj(q1) + conj(q2) + conj(q3) + conj(q4))*sin(conj(q1))*cos(q1 + q2 + q3 + q4)*cos(q1 + q2)*conj(L1)*conj(L4) - 2*L2*L4*sin(conj(q1) + conj(q2) + conj(q3) + conj(q4))*cos(conj(q1))*cos(q1 + q2 + q3 + q4)*cos(q1 + q2)*conj(L1)*conj(L4) + 2*L2*L4*cos(conj(q1) + conj(q2) + conj(q3) + conj(q4))*cos(conj(q1) + conj(q2) + conj(q3))*cos(q1 + q2 + q3 + q4)*conj(L3)*conj(L4)*sin(q1 + q2) - 2*L2*L4*cos(conj(q1) + conj(q2) + conj(q3) + conj(q4))*cos(conj(q1) + conj(q2) + conj(q3))*sin(q1 + q2 + q3 + q4)*cos(q1 + q2)*conj(L3)*conj(L4) + 2*L2*L4*cos(conj(q1) + conj(q2) + conj(q3) + conj(q4))*sin(conj(q1) + conj(q2) + conj(q3))*cos(q1 + q2 + q3 + q4)*cos(q1 + q2)*conj(L3)*conj(L4) - 2*L2*L4*sin(conj(q1) + conj(q2) + conj(q3) + conj(q4))*cos(conj(q1) + conj(q2) + conj(q3))*cos(q1 + q2 + q3 + q4)*cos(q1 + q2)*conj(L3)*conj(L4) + L1*L3*cos(q1 + q2 + q3)*sin(conj(q1) + conj(q2) + conj(q3) + conj(q4))*sin(conj(q1) + conj(q2))*conj(L2)*conj(L4)*sin(q1) - L1*L3*sin(conj(q1) + conj(q2) + conj(q3) + conj(q4))*sin(q1 + q2 + q3)*sin(conj(q1) + conj(q2))*conj(L2)*conj(L4)*cos(q1) + 2*L2*L4*cos(conj(q1) + conj(q2) + conj(q3) + conj(q4))*sin(conj(q1))*sin(q1 + q2 + q3 + q4)*conj(L1)*conj(L4)*sin(q1 + q2) - 2*L2*L4*sin(conj(q1) + conj(q2) + conj(q3) + conj(q4))*cos(conj(q1))*sin(q1 + q2 + q3 + q4)*conj(L1)*conj(L4)*sin(q1 + q2) + 2*L2*L4*sin(conj(q1) + conj(q2) + conj(q3) + conj(q4))*sin(conj(q1))*cos(q1 + q2 + q3 + q4)*conj(L1)*conj(L4)*sin(q1 + q2) - 2*L2*L4*sin(conj(q1) + conj(q2) + conj(q3) + conj(q4))*sin(conj(q1))*sin(q1 + q2 + q3 + q4)*cos(q1 + q2)*conj(L1)*conj(L4)))/(L1*L3*cos(q1 + q2 + q3)*sin(conj(q1))*cos(conj(q1) + conj(q2))*conj(L1)*conj(L2)*sin(q1) - L1*L3*cos(q1 + q2 + q3)*cos(conj(q1))*sin(conj(q1) + conj(q2))*conj(L1)*conj(L2)*sin(q1) + L1*L3*sin(q1 + q2 + q3)*cos(conj(q1))*sin(conj(q1) + conj(q2))*conj(L1)*conj(L2)*cos(q1) - L1*L3*sin(q1 + q2 + q3)*sin(conj(q1))*cos(conj(q1) + conj(q2))*conj(L1)*conj(L2)*cos(q1) + L1*L3*cos(q1 + q2 + q3)*cos(conj(q1) + conj(q2) + conj(q3))*sin(conj(q1) + conj(q2))*conj(L2)*conj(L3)*sin(q1) - L1*L3*cos(q1 + q2 + q3)*sin(conj(q1) + conj(q2) + conj(q3))*cos(conj(q1) + conj(q2))*conj(L2)*conj(L3)*sin(q1) - L1*L3*sin(q1 + q2 + q3)*cos(conj(q1) + conj(q2) + conj(q3))*sin(conj(q1) + conj(q2))*conj(L2)*conj(L3)*cos(q1) + L1*L3*sin(q1 + q2 + q3)*sin(conj(q1) + conj(q2) + conj(q3))*cos(conj(q1) + conj(q2))*conj(L2)*conj(L3)*cos(q1) - L2*L4*cos(conj(q1))*sin(conj(q1) + conj(q2) + conj(q3))*cos(q1 + q2 + q3 + q4)*conj(L1)*conj(L3)*sin(q1 + q2) + L2*L4*cos(conj(q1))*sin(conj(q1) + conj(q2) + conj(q3))*sin(q1 + q2 + q3 + q4)*cos(q1 + q2)*conj(L1)*conj(L3) + L2*L4*cos(conj(q1) + conj(q2) + conj(q3))*sin(conj(q1))*cos(q1 + q2 + q3 + q4)*conj(L1)*conj(L3)*sin(q1 + q2) - L2*L4*cos(conj(q1) + conj(q2) + conj(q3))*sin(conj(q1))*sin(q1 + q2 + q3 + q4)*cos(q1 + q2)*conj(L1)*conj(L3) + 3*L1*L4*cos(conj(q1) + conj(q2) + conj(q3) + conj(q4))*sin(conj(q1))*cos(q1 + q2 + q3 + q4)*conj(L1)*conj(L4)*sin(q1) - 3*L1*L4*cos(conj(q1) + conj(q2) + conj(q3) + conj(q4))*sin(conj(q1))*sin(q1 + q2 + q3 + q4)*conj(L1)*conj(L4)*cos(q1) - 3*L1*L4*sin(conj(q1) + conj(q2) + conj(q3) + conj(q4))*cos(conj(q1))*cos(q1 + q2 + q3 + q4)*conj(L1)*conj(L4)*sin(q1) + 3*L1*L4*sin(conj(q1) + conj(q2) + conj(q3) + conj(q4))*cos(conj(q1))*sin(q1 + q2 + q3 + q4)*conj(L1)*conj(L4)*cos(q1) + 4*L2*L4*cos(conj(q1) + conj(q2) + conj(q3) + conj(q4))*sin(conj(q1) + conj(q2))*cos(q1 + q2 + q3 + q4)*conj(L2)*conj(L4)*sin(q1 + q2) - 4*L2*L4*cos(conj(q1) + conj(q2) + conj(q3) + conj(q4))*sin(conj(q1) + conj(q2))*sin(q1 + q2 + q3 + q4)*cos(q1 + q2)*conj(L2)*conj(L4) - 4*L2*L4*sin(conj(q1) + conj(q2) + conj(q3) + conj(q4))*cos(conj(q1) + conj(q2))*cos(q1 + q2 + q3 + q4)*conj(L2)*conj(L4)*sin(q1 + q2) + 4*L2*L4*sin(conj(q1) + conj(q2) + conj(q3) + conj(q4))*cos(conj(q1) + conj(q2))*sin(q1 + q2 + q3 + q4)*cos(q1 + q2)*conj(L2)*conj(L4) + L1*L4*cos(conj(q1) + conj(q2) + conj(q3) + conj(q4))*sin(conj(q1) + conj(q2) + conj(q3))*cos(q1 + q2 + q3 + q4)*conj(L3)*conj(L4)*sin(q1) - L1*L4*cos(conj(q1) + conj(q2) + conj(q3) + conj(q4))*sin(conj(q1) + conj(q2) + conj(q3))*sin(q1 + q2 + q3 + q4)*conj(L3)*conj(L4)*cos(q1) - L1*L4*sin(conj(q1) + conj(q2) + conj(q3) + conj(q4))*cos(conj(q1) + conj(q2) + conj(q3))*cos(q1 + q2 + q3 + q4)*conj(L3)*conj(L4)*sin(q1) + L1*L4*sin(conj(q1) + conj(q2) + conj(q3) + conj(q4))*cos(conj(q1) + conj(q2) + conj(q3))*sin(q1 + q2 + q3 + q4)*conj(L3)*conj(L4)*cos(q1) + L1*L2*cos(conj(q1) + conj(q2) + conj(q3) + conj(q4))*sin(conj(q1))*cos(q1 + q2)*conj(L1)*conj(L4)*sin(q1) - L1*L2*cos(conj(q1) + conj(q2) + conj(q3) + conj(q4))*sin(conj(q1))*conj(L1)*conj(L4)*sin(q1 + q2)*cos(q1) - L1*L2*sin(conj(q1) + conj(q2) + conj(q3) + conj(q4))*cos(conj(q1))*cos(q1 + q2)*conj(L1)*conj(L4)*sin(q1) + L1*L2*sin(conj(q1) + conj(q2) + conj(q3) + conj(q4))*cos(conj(q1))*conj(L1)*conj(L4)*sin(q1 + q2)*cos(q1) - 2*L1*L4*cos(conj(q1))*sin(conj(q1) + conj(q2) + conj(q3))*cos(q1 + q2 + q3 + q4)*conj(L1)*conj(L3)*sin(q1) + 2*L1*L4*cos(conj(q1))*sin(conj(q1) + conj(q2) + conj(q3))*sin(q1 + q2 + q3 + q4)*conj(L1)*conj(L3)*cos(q1) + 2*L1*L4*cos(conj(q1) + conj(q2) + conj(q3))*sin(conj(q1))*cos(q1 + q2 + q3 + q4)*conj(L1)*conj(L3)*sin(q1) - 2*L1*L4*cos(conj(q1) + conj(q2) + conj(q3))*sin(conj(q1))*sin(q1 + q2 + q3 + q4)*conj(L1)*conj(L3)*cos(q1) + 2*L2*L4*cos(conj(q1) + conj(q2) + conj(q3))*sin(conj(q1) + conj(q2))*cos(q1 + q2 + q3 + q4)*conj(L2)*conj(L3)*sin(q1 + q2) - 2*L2*L4*cos(conj(q1) + conj(q2) + conj(q3))*sin(conj(q1) + conj(q2))*sin(q1 + q2 + q3 + q4)*cos(q1 + q2)*conj(L2)*conj(L3) - 2*L2*L4*sin(conj(q1) + conj(q2) + conj(q3))*cos(conj(q1) + conj(q2))*cos(q1 + q2 + q3 + q4)*conj(L2)*conj(L3)*sin(q1 + q2) + 2*L2*L4*sin(conj(q1) + conj(q2) + conj(q3))*cos(conj(q1) + conj(q2))*sin(q1 + q2 + q3 + q4)*cos(q1 + q2)*conj(L2)*conj(L3) + 2*L1*L4*cos(conj(q1) + conj(q2) + conj(q3) + conj(q4))*sin(conj(q1) + conj(q2))*cos(q1 + q2 + q3 + q4)*conj(L2)*conj(L4)*sin(q1) - 2*L1*L4*cos(conj(q1) + conj(q2) + conj(q3) + conj(q4))*sin(conj(q1) + conj(q2))*sin(q1 + q2 + q3 + q4)*conj(L2)*conj(L4)*cos(q1) - 2*L1*L4*sin(conj(q1) + conj(q2) + conj(q3) + conj(q4))*cos(conj(q1) + conj(q2))*cos(q1 + q2 + q3 + q4)*conj(L2)*conj(L4)*sin(q1) + 2*L1*L4*sin(conj(q1) + conj(q2) + conj(q3) + conj(q4))*cos(conj(q1) + conj(q2))*sin(q1 + q2 + q3 + q4)*conj(L2)*conj(L4)*cos(q1) - L3*L4*cos(conj(q1) + conj(q2) + conj(q3) + conj(q4))*cos(q1 + q2 + q3)*sin(conj(q1))*sin(q1 + q2 + q3 + q4)*conj(L1)*conj(L4) + L3*L4*cos(conj(q1) + conj(q2) + conj(q3) + conj(q4))*sin(q1 + q2 + q3)*sin(conj(q1))*cos(q1 + q2 + q3 + q4)*conj(L1)*conj(L4) + L3*L4*cos(q1 + q2 + q3)*sin(conj(q1) + conj(q2) + conj(q3) + conj(q4))*cos(conj(q1))*sin(q1 + q2 + q3 + q4)*conj(L1)*conj(L4) - L3*L4*sin(conj(q1) + conj(q2) + conj(q3) + conj(q4))*sin(q1 + q2 + q3)*cos(conj(q1))*cos(q1 + q2 + q3 + q4)*conj(L1)*conj(L4) - L1*L2*cos(conj(q1))*sin(conj(q1) + conj(q2) + conj(q3))*cos(q1 + q2)*conj(L1)*conj(L3)*sin(q1) + L1*L2*cos(conj(q1))*sin(conj(q1) + conj(q2) + conj(q3))*conj(L1)*conj(L3)*sin(q1 + q2)*cos(q1) + L1*L2*cos(conj(q1) + conj(q2) + conj(q3))*sin(conj(q1))*cos(q1 + q2)*conj(L1)*conj(L3)*sin(q1) - L1*L2*cos(conj(q1) + conj(q2) + conj(q3))*sin(conj(q1))*conj(L1)*conj(L3)*sin(q1 + q2)*cos(q1) - 3*L3*L4*cos(conj(q1) + conj(q2) + conj(q3) + conj(q4))*cos(q1 + q2 + q3)*sin(conj(q1) + conj(q2) + conj(q3))*sin(q1 + q2 + q3 + q4)*conj(L3)*conj(L4) + 3*L3*L4*cos(conj(q1) + conj(q2) + conj(q3) + conj(q4))*sin(q1 + q2 + q3)*sin(conj(q1) + conj(q2) + conj(q3))*cos(q1 + q2 + q3 + q4)*conj(L3)*conj(L4) + 3*L3*L4*cos(q1 + q2 + q3)*sin(conj(q1) + conj(q2) + conj(q3) + conj(q4))*cos(conj(q1) + conj(q2) + conj(q3))*sin(q1 + q2 + q3 + q4)*conj(L3)*conj(L4) - 3*L3*L4*sin(conj(q1) + conj(q2) + conj(q3) + conj(q4))*sin(q1 + q2 + q3)*cos(conj(q1) + conj(q2) + conj(q3))*cos(q1 + q2 + q3 + q4)*conj(L3)*conj(L4) - L1*L4*cos(conj(q1))*sin(conj(q1) + conj(q2))*cos(q1 + q2 + q3 + q4)*conj(L1)*conj(L2)*sin(q1) + L1*L4*cos(conj(q1))*sin(conj(q1) + conj(q2))*sin(q1 + q2 + q3 + q4)*conj(L1)*conj(L2)*cos(q1) + L1*L4*sin(conj(q1))*cos(conj(q1) + conj(q2))*cos(q1 + q2 + q3 + q4)*conj(L1)*conj(L2)*sin(q1) - L1*L4*sin(conj(q1))*cos(conj(q1) + conj(q2))*sin(q1 + q2 + q3 + q4)*conj(L1)*conj(L2)*cos(q1) + L1*L4*cos(conj(q1) + conj(q2) + conj(q3))*sin(conj(q1) + conj(q2))*cos(q1 + q2 + q3 + q4)*conj(L2)*conj(L3)*sin(q1) - L1*L4*cos(conj(q1) + conj(q2) + conj(q3))*sin(conj(q1) + conj(q2))*sin(q1 + q2 + q3 + q4)*conj(L2)*conj(L3)*cos(q1) - L1*L4*sin(conj(q1) + conj(q2) + conj(q3))*cos(conj(q1) + conj(q2))*cos(q1 + q2 + q3 + q4)*conj(L2)*conj(L3)*sin(q1) + L1*L4*sin(conj(q1) + conj(q2) + conj(q3))*cos(conj(q1) + conj(q2))*sin(q1 + q2 + q3 + q4)*conj(L2)*conj(L3)*cos(q1) + L2*L3*cos(conj(q1) + conj(q2) + conj(q3) + conj(q4))*cos(q1 + q2 + q3)*sin(conj(q1))*conj(L1)*conj(L4)*sin(q1 + q2) - L2*L3*cos(conj(q1) + conj(q2) + conj(q3) + conj(q4))*sin(q1 + q2 + q3)*sin(conj(q1))*cos(q1 + q2)*conj(L1)*conj(L4) - L2*L3*cos(q1 + q2 + q3)*sin(conj(q1) + conj(q2) + conj(q3) + conj(q4))*cos(conj(q1))*conj(L1)*conj(L4)*sin(q1 + q2) + L2*L3*sin(conj(q1) + conj(q2) + conj(q3) + conj(q4))*sin(q1 + q2 + q3)*cos(conj(q1))*cos(q1 + q2)*conj(L1)*conj(L4) - L1*L2*cos(conj(q1))*sin(conj(q1) + conj(q2))*cos(q1 + q2)*conj(L1)*conj(L2)*sin(q1) + L1*L2*cos(conj(q1))*sin(conj(q1) + conj(q2))*conj(L1)*conj(L2)*sin(q1 + q2)*cos(q1) + L1*L2*sin(conj(q1))*cos(conj(q1) + conj(q2))*cos(q1 + q2)*conj(L1)*conj(L2)*sin(q1) - L1*L2*sin(conj(q1))*cos(conj(q1) + conj(q2))*conj(L1)*conj(L2)*sin(q1 + q2)*cos(q1) - 2*L3*L4*cos(conj(q1) + conj(q2) + conj(q3) + conj(q4))*cos(q1 + q2 + q3)*sin(conj(q1) + conj(q2))*sin(q1 + q2 + q3 + q4)*conj(L2)*conj(L4) + 2*L3*L4*cos(conj(q1) + conj(q2) + conj(q3) + conj(q4))*sin(q1 + q2 + q3)*sin(conj(q1) + conj(q2))*cos(q1 + q2 + q3 + q4)*conj(L2)*conj(L4) + 2*L3*L4*cos(q1 + q2 + q3)*sin(conj(q1) + conj(q2) + conj(q3) + conj(q4))*cos(conj(q1) + conj(q2))*sin(q1 + q2 + q3 + q4)*conj(L2)*conj(L4) - 2*L3*L4*sin(conj(q1) + conj(q2) + conj(q3) + conj(q4))*sin(q1 + q2 + q3)*cos(conj(q1) + conj(q2))*cos(q1 + q2 + q3 + q4)*conj(L2)*conj(L4) - L2*L3*cos(q1 + q2 + q3)*cos(conj(q1))*sin(conj(q1) + conj(q2) + conj(q3))*conj(L1)*conj(L3)*sin(q1 + q2) + L2*L3*cos(q1 + q2 + q3)*cos(conj(q1) + conj(q2) + conj(q3))*sin(conj(q1))*conj(L1)*conj(L3)*sin(q1 + q2) + L2*L3*sin(q1 + q2 + q3)*cos(conj(q1))*sin(conj(q1) + conj(q2) + conj(q3))*cos(q1 + q2)*conj(L1)*conj(L3) - L2*L3*sin(q1 + q2 + q3)*cos(conj(q1) + conj(q2) + conj(q3))*sin(conj(q1))*cos(q1 + q2)*conj(L1)*conj(L3) + 2*L1*L3*cos(conj(q1) + conj(q2) + conj(q3) + conj(q4))*cos(q1 + q2 + q3)*sin(conj(q1))*conj(L1)*conj(L4)*sin(q1) - 2*L1*L3*cos(conj(q1) + conj(q2) + conj(q3) + conj(q4))*sin(q1 + q2 + q3)*sin(conj(q1))*conj(L1)*conj(L4)*cos(q1) - 2*L1*L3*cos(q1 + q2 + q3)*sin(conj(q1) + conj(q2) + conj(q3) + conj(q4))*cos(conj(q1))*conj(L1)*conj(L4)*sin(q1) + 2*L1*L3*sin(conj(q1) + conj(q2) + conj(q3) + conj(q4))*sin(q1 + q2 + q3)*cos(conj(q1))*conj(L1)*conj(L4)*cos(q1) + 2*L2*L3*cos(conj(q1) + conj(q2) + conj(q3) + conj(q4))*cos(q1 + q2 + q3)*sin(conj(q1) + conj(q2))*conj(L2)*conj(L4)*sin(q1 + q2) - 2*L2*L3*cos(conj(q1) + conj(q2) + conj(q3) + conj(q4))*sin(q1 + q2 + q3)*sin(conj(q1) + conj(q2))*cos(q1 + q2)*conj(L2)*conj(L4) - 2*L2*L3*cos(q1 + q2 + q3)*sin(conj(q1) + conj(q2) + conj(q3) + conj(q4))*cos(conj(q1) + conj(q2))*conj(L2)*conj(L4)*sin(q1 + q2) + 2*L2*L3*sin(conj(q1) + conj(q2) + conj(q3) + conj(q4))*sin(q1 + q2 + q3)*cos(conj(q1) + conj(q2))*cos(q1 + q2)*conj(L2)*conj(L4) - 2*L1*L3*cos(q1 + q2 + q3)*cos(conj(q1))*sin(conj(q1) + conj(q2) + conj(q3))*conj(L1)*conj(L3)*sin(q1) + 2*L1*L3*cos(q1 + q2 + q3)*cos(conj(q1) + conj(q2) + conj(q3))*sin(conj(q1))*conj(L1)*conj(L3)*sin(q1) + 2*L1*L3*sin(q1 + q2 + q3)*cos(conj(q1))*sin(conj(q1) + conj(q2) + conj(q3))*conj(L1)*conj(L3)*cos(q1) - 2*L1*L3*sin(q1 + q2 + q3)*cos(conj(q1) + conj(q2) + conj(q3))*sin(conj(q1))*conj(L1)*conj(L3)*cos(q1) + 2*L2*L3*cos(q1 + q2 + q3)*cos(conj(q1) + conj(q2) + conj(q3))*sin(conj(q1) + conj(q2))*conj(L2)*conj(L3)*sin(q1 + q2) - 2*L2*L3*cos(q1 + q2 + q3)*sin(conj(q1) + conj(q2) + conj(q3))*cos(conj(q1) + conj(q2))*conj(L2)*conj(L3)*sin(q1 + q2) - 2*L2*L3*sin(q1 + q2 + q3)*cos(conj(q1) + conj(q2) + conj(q3))*sin(conj(q1) + conj(q2))*cos(q1 + q2)*conj(L2)*conj(L3) + 2*L2*L3*sin(q1 + q2 + q3)*sin(conj(q1) + conj(q2) + conj(q3))*cos(conj(q1) + conj(q2))*cos(q1 + q2)*conj(L2)*conj(L3) + L1*L3*cos(conj(q1) + conj(q2) + conj(q3) + conj(q4))*cos(q1 + q2 + q3)*sin(conj(q1) + conj(q2))*conj(L2)*conj(L4)*sin(q1) - L1*L3*cos(conj(q1) + conj(q2) + conj(q3) + conj(q4))*sin(q1 + q2 + q3)*sin(conj(q1) + conj(q2))*conj(L2)*conj(L4)*cos(q1) - L1*L3*cos(q1 + q2 + q3)*sin(conj(q1) + conj(q2) + conj(q3) + conj(q4))*cos(conj(q1) + conj(q2))*conj(L2)*conj(L4)*sin(q1) + L1*L3*sin(conj(q1) + conj(q2) + conj(q3) + conj(q4))*sin(q1 + q2 + q3)*cos(conj(q1) + conj(q2))*conj(L2)*conj(L4)*cos(q1) + 2*L2*L4*cos(conj(q1) + conj(q2) + conj(q3) + conj(q4))*sin(conj(q1))*cos(q1 + q2 + q3 + q4)*conj(L1)*conj(L4)*sin(q1 + q2) - 2*L2*L4*cos(conj(q1) + conj(q2) + conj(q3) + conj(q4))*sin(conj(q1))*sin(q1 + q2 + q3 + q4)*cos(q1 + q2)*conj(L1)*conj(L4) - 2*L2*L4*sin(conj(q1) + conj(q2) + conj(q3) + conj(q4))*cos(conj(q1))*cos(q1 + q2 + q3 + q4)*conj(L1)*conj(L4)*sin(q1 + q2) + 2*L2*L4*sin(conj(q1) + conj(q2) + conj(q3) + conj(q4))*cos(conj(q1))*sin(q1 + q2 + q3 + q4)*cos(q1 + q2)*conj(L1)*conj(L4) + 2*L2*L4*cos(conj(q1) + conj(q2) + conj(q3) + conj(q4))*sin(conj(q1) + conj(q2) + conj(q3))*cos(q1 + q2 + q3 + q4)*conj(L3)*conj(L4)*sin(q1 + q2) - 2*L2*L4*cos(conj(q1) + conj(q2) + conj(q3) + conj(q4))*sin(conj(q1) + conj(q2) + conj(q3))*sin(q1 + q2 + q3 + q4)*cos(q1 + q2)*conj(L3)*conj(L4) - 2*L2*L4*sin(conj(q1) + conj(q2) + conj(q3) + conj(q4))*cos(conj(q1) + conj(q2) + conj(q3))*cos(q1 + q2 + q3 + q4)*conj(L3)*conj(L4)*sin(q1 + q2) + 2*L2*L4*sin(conj(q1) + conj(q2) + conj(q3) + conj(q4))*cos(conj(q1) + conj(q2) + conj(q3))*sin(q1 + q2 + q3 + q4)*cos(q1 + q2)*conj(L3)*conj(L4))^0.5000;
%%%
aux = -1*[aux11; aux21; aux31; aux41];
